simulink model "switch_inductor_system"  (R2025b)
settings: Solver=ode23t  StartTime=0.0  StopTime=10e-6  MaxStep=1e-8  RelTol=1e-4
libraries: fl_lib x93, nesl_utility x82, eeGeneralControl x28, batteryecm_lib x17, eePwmGenerator x11, slpidlib x9, simulink x2, slctrl_fre x1
(part 1 of 3)
settings Model: Creator=wjy22  LastModifiedBy=wjy22

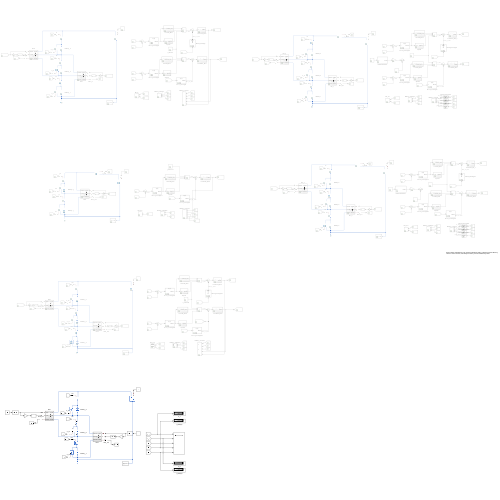
[thumbnail: Simulink's stored preview of the top-level diagram]
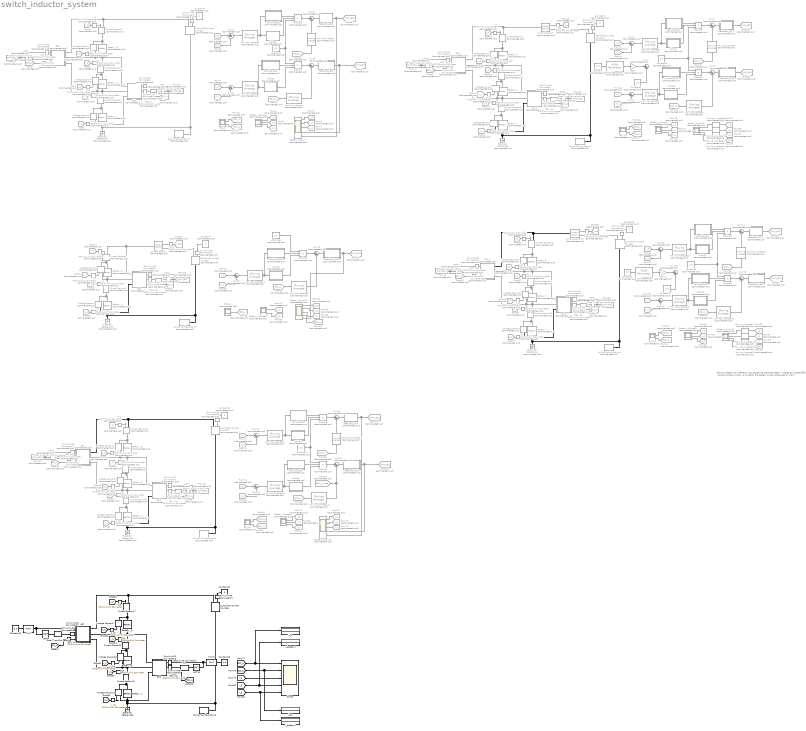
== system switch_inductor_system ==
  note: Same voltage with different inner resistance, Balance battery voltage at highest efficiency inductor current window, and satisfy the battery current scheduled by SOH.
  Alpha1 : Subsystem  Commented=on
  Alpha2 : Subsystem  Commented=on
  Alpha3 : Subsystem  Commented=on
  Alpha4 : Subsystem  Commented=on
  Alpha5 : Subsystem  Commented=on
  Alpha6 : Subsystem  Commented=on
  Alpha7 : Subsystem  Commented=on
  Alpha8 : Subsystem  Commented=on
  Alpha9 : Subsystem  Commented=on
  BC1 : Subsystem  Commented=on
  BC1_IL{,1..4} (5 alike) : nesl_utility/PS-Simulink Converter  Commented=on  PhysicalDomain=network_engine_domain  SubClassName=ps_output  LeftPortType=input  RightPortType=output  PseudoPeriodic=off  Frequencies=[]  VectorFormat=inherit  Unit=inherit  AffineConversion=off
  BC1_IL5 : nesl_utility/PS-Simulink Converter  PhysicalDomain=network_engine_domain  SubClassName=ps_output  LeftPortType=input  RightPortType=output  PseudoPeriodic=off  Frequencies=[]  VectorFormat=inherit  Unit=inherit  AffineConversion=off
  BC2 : Subsystem  Commented=on
  BC2_IL{,1..3} (4 alike) : nesl_utility/PS-Simulink Converter  Commented=on  PhysicalDomain=network_engine_domain  SubClassName=ps_output  LeftPortType=input  RightPortType=output  PseudoPeriodic=off  Frequencies=[]  VectorFormat=inherit  Unit=inherit  AffineConversion=off
  BC2_IL4 : nesl_utility/PS-Simulink Converter  PhysicalDomain=network_engine_domain  SubClassName=ps_output  LeftPortType=input  RightPortType=output  PseudoPeriodic=off  Frequencies=[]  VectorFormat=inherit  Unit=inherit  AffineConversion=off
  BC3 : Subsystem  Commented=on
  BC4 : Subsystem  Commented=on
  BC5 : Subsystem  Commented=on
  BC6 : Subsystem
  BC7 : Subsystem
  BC_1 : Subsystem  Commented=on
  BC_2 : Subsystem  Commented=on
  BC_3 : Subsystem  Commented=on
  BC_4 : Subsystem  Commented=on
  BC_IL{,1,3..4} (4 alike) : Scope  Commented=on  NumInputPorts=2
      BC_IL settings: ActiveDisplayYMinimum=0.30113223762513219  ActiveDisplayYMaximum=0.30789063396141053  DataLoggingVariableName=ScopeData4
      BC_IL1 settings: ActiveDisplayYMinimum=-0.37448035272574393  ActiveDisplayYMaximum=-0.29986535447261758
      BC_IL3 settings: ActiveDisplayYMinimum=-0.37448035272574393  ActiveDisplayYMaximum=-0.29986535447261758  DataLoggingVariableName=ScopeData14
      BC_IL4 settings: ActiveDisplayYMinimum=0.30113223762513219  ActiveDisplayYMaximum=0.30789063396141053  DataLoggingVariableName=ScopeData17
  BC_IL2 : Scope  Commented=on
      settings: ActiveDisplayYMinimum=-0.43402408027628592  ActiveDisplayYMaximum=0.45876699221950035  DataLoggingVariableName=ScopeData6
  Battery 1 : batteryecm_lib/Battery  Commented=on  Vnom=4.2 V  prm_dir=simscape.enum.battery.prm_dir.disabled  R1_dis=2 Ohm  R1_ch=2 Ohm  R1=0.0075 Ohm  prm_AH=simscape.enum.battery.prm_AH.finite  AH=0.0026 A*hr  V1=3.7 V  AH1=0.00143 A*hr  prm_R2=simscape.enum.battery.prm_R2.disabled  R2=2000 Ohm  Tmeas=298.15 K  charge_measurement_port=simscape.enum.battery.enable.no  prm_dyn=simscape.enum.battery.prm_dyn.off  Rp1=0.005 Ohm  tau1=30 s  Rp2=0.005 Ohm  tau2=30 s  Rp3=0.005 Ohm  tau3=30 s  Rp4=0.005 Ohm  tau4=30 s  Rp5=0.005 Ohm  tau5=30 s  prm_fade=simscape.enum.battery.prm_fade.disabled  N_fade=100  AH_fade=45 A*hr  R1_fade=2.02 Ohm  R1_ch_fade=2.02 Ohm  V1_fade=10.35 V  prm_age=simscape.enum.battery.prm_age.disabled  prm_age_OCV=simscape.enum.battery.prm_age_OCV.OCV  OCV_age=0.9  SOC_age=60  Tmeas_age=298.15 K  delta_time_age_vec=[0] d  temperature_age_vec=[273] K  OCV_scaling_age=2.2134e6  OCV_offset_age=1.632e6  temp_exp_age=0.515833569 V  t_exp_age=0.75  Vnom_T2=12 V  R1_T2=2.2 Ohm  R1_T2_dis=2.2 Ohm  R1_T2_ch=2.2 Ohm  V1_T2=11.4 V  R2_T2=2200 Ohm  Rp1_T2=0.005 Ohm  tau1_T2=30 s  Rp2_T2=0.005 Ohm  tau2_T2=30 s  Rp3_T2=0.005 Ohm  tau3_T2=30 s  Rp4_T2=0.005 Ohm  tau4_T2=30 s  Rp5_T2=0.005 Ohm  tau5_T2=30 s  Tmeas2=273.15 K  thermal_port=simscape.enum.thermaleffects.omit  thermal_mass=30000 J/K  i_specify=off  i_priority=None  i=0 A  i_nominal_specify=off  i_nominal_value=1  i_nominal_unit=A  v_specify=on  v_priority=High  v=3.8 V  v_nominal_specify=off  v_nominal_value=1  v_nominal_unit=V  charge_specify=on  charge_priority=None  charge=0.001072 A*hr  charge_nominal_specify=off  charge_nominal_value=1  charge_nominal_unit=A*hr  num_cycles_specify=off  num_cycles_priority=High  num_cycles=0  num_cycles_nominal_specify=off  num_cycles_nominal_value=1  num_cycles_nominal_unit=1  temperature_specify=off  temperature_priority=High  temperature=298.15 K  temperature_nominal_specify=off  temperature_nominal_value=1  temperature_nominal_unit=K
      settings: LibrarySourceBlock=batt_lib/Cells/Battery
  Battery 1_ : batteryecm_lib/Battery  Commented=on  Vnom=4.2 V  prm_dir=simscape.enum.battery.prm_dir.disabled  R1_dis=2 Ohm  R1_ch=2 Ohm  R1=0.0065 Ohm  prm_AH=simscape.enum.battery.prm_AH.finite  AH=0.0026 A*hr  V1=3.7 V  AH1=0.00143 A*hr  prm_R2=simscape.enum.battery.prm_R2.disabled  R2=2000 Ohm  Tmeas=298.15 K  charge_measurement_port=simscape.enum.battery.enable.no  prm_dyn=simscape.enum.battery.prm_dyn.off  Rp1=0.005 Ohm  tau1=30 s  Rp2=0.005 Ohm  tau2=30 s  Rp3=0.005 Ohm  tau3=30 s  Rp4=0.005 Ohm  tau4=30 s  Rp5=0.005 Ohm  tau5=30 s  prm_fade=simscape.enum.battery.prm_fade.disabled  N_fade=100  AH_fade=45 A*hr  R1_fade=2.02 Ohm  R1_ch_fade=2.02 Ohm  V1_fade=10.35 V  prm_age=simscape.enum.battery.prm_age.disabled  prm_age_OCV=simscape.enum.battery.prm_age_OCV.OCV  OCV_age=0.9  SOC_age=60  Tmeas_age=298.15 K  delta_time_age_vec=[0] d  temperature_age_vec=[273] K  OCV_scaling_age=2.2134e6  OCV_offset_age=1.632e6  temp_exp_age=0.515833569 V  t_exp_age=0.75  Vnom_T2=12 V  R1_T2=2.2 Ohm  R1_T2_dis=2.2 Ohm  R1_T2_ch=2.2 Ohm  V1_T2=11.4 V  R2_T2=2200 Ohm  Rp1_T2=0.005 Ohm  tau1_T2=30 s  Rp2_T2=0.005 Ohm  tau2_T2=30 s  Rp3_T2=0.005 Ohm  tau3_T2=30 s  Rp4_T2=0.005 Ohm  tau4_T2=30 s  Rp5_T2=0.005 Ohm  tau5_T2=30 s  Tmeas2=273.15 K  thermal_port=simscape.enum.thermaleffects.omit  thermal_mass=30000 J/K  i_specify=off  i_priority=None  i=0 A  i_nominal_specify=off  i_nominal_value=1  i_nominal_unit=A  v_specify=on  v_priority=High  v=4 V  v_nominal_specify=off  v_nominal_value=1  v_nominal_unit=V  charge_specify=on  charge_priority=None  charge=0.001072 A*hr  charge_nominal_specify=off  charge_nominal_value=1  charge_nominal_unit=A*hr  num_cycles_specify=off  num_cycles_priority=High  num_cycles=0  num_cycles_nominal_specify=off  num_cycles_nominal_value=1  num_cycles_nominal_unit=1  temperature_specify=off  temperature_priority=High  temperature=298.15 K  temperature_nominal_specify=off  temperature_nominal_value=1  temperature_nominal_unit=K
      settings: LibrarySourceBlock=batt_lib/Cells/Battery
  Battery 2 : batteryecm_lib/Battery  Commented=on  Vnom=4.2 V  prm_dir=simscape.enum.battery.prm_dir.disabled  R1_dis=2 Ohm  R1_ch=2 Ohm  R1=0.0065 Ohm  prm_AH=simscape.enum.battery.prm_AH.finite  AH=0.0026 A*hr  V1=3.7 V  AH1=0.00143 A*hr  prm_R2=simscape.enum.battery.prm_R2.disabled  R2=2000 Ohm  Tmeas=298.15 K  charge_measurement_port=simscape.enum.battery.enable.no  prm_dyn=simscape.enum.battery.prm_dyn.off  Rp1=0.005 Ohm  tau1=30 s  Rp2=0.005 Ohm  tau2=30 s  Rp3=0.005 Ohm  tau3=30 s  Rp4=0.005 Ohm  tau4=30 s  Rp5=0.005 Ohm  tau5=30 s  prm_fade=simscape.enum.battery.prm_fade.disabled  N_fade=100  AH_fade=45 A*hr  R1_fade=2.02 Ohm  R1_ch_fade=2.02 Ohm  V1_fade=10.35 V  prm_age=simscape.enum.battery.prm_age.disabled  prm_age_OCV=simscape.enum.battery.prm_age_OCV.OCV  OCV_age=0.9  SOC_age=60  Tmeas_age=298.15 K  delta_time_age_vec=[0] d  temperature_age_vec=[273] K  OCV_scaling_age=2.2134e6  OCV_offset_age=1.632e6  temp_exp_age=0.515833569 V  t_exp_age=0.75  Vnom_T2=12 V  R1_T2=2.2 Ohm  R1_T2_dis=2.2 Ohm  R1_T2_ch=2.2 Ohm  V1_T2=11.4 V  R2_T2=2200 Ohm  Rp1_T2=0.005 Ohm  tau1_T2=30 s  Rp2_T2=0.005 Ohm  tau2_T2=30 s  Rp3_T2=0.005 Ohm  tau3_T2=30 s  Rp4_T2=0.005 Ohm  tau4_T2=30 s  Rp5_T2=0.005 Ohm  tau5_T2=30 s  Tmeas2=273.15 K  thermal_port=simscape.enum.thermaleffects.omit  thermal_mass=30000 J/K  i_specify=off  i_priority=None  i=0 A  i_nominal_specify=off  i_nominal_value=1  i_nominal_unit=A  v_specify=on  v_priority=High  v=4 V  v_nominal_specify=off  v_nominal_value=1  v_nominal_unit=V  charge_specify=on  charge_priority=None  charge=0.001588 A*hr  charge_nominal_specify=off  charge_nominal_value=1  charge_nominal_unit=A*hr  num_cycles_specify=off  num_cycles_priority=High  num_cycles=0  num_cycles_nominal_specify=off  num_cycles_nominal_value=1  num_cycles_nominal_unit=1  temperature_specify=off  temperature_priority=High  temperature=298.15 K  temperature_nominal_specify=off  temperature_nominal_value=1  temperature_nominal_unit=K
      settings: LibrarySourceBlock=batt_lib/Cells/Battery
  Battery 2_ : batteryecm_lib/Battery  Commented=on  Vnom=4.2 V  prm_dir=simscape.enum.battery.prm_dir.disabled  R1_dis=2 Ohm  R1_ch=2 Ohm  R1=0.0065 Ohm  prm_AH=simscape.enum.battery.prm_AH.finite  AH=0.0026 A*hr  V1=3.7 V  AH1=0.00143 A*hr  prm_R2=simscape.enum.battery.prm_R2.disabled  R2=2000 Ohm  Tmeas=298.15 K  charge_measurement_port=simscape.enum.battery.enable.no  prm_dyn=simscape.enum.battery.prm_dyn.off  Rp1=0.005 Ohm  tau1=30 s  Rp2=0.005 Ohm  tau2=30 s  Rp3=0.005 Ohm  tau3=30 s  Rp4=0.005 Ohm  tau4=30 s  Rp5=0.005 Ohm  tau5=30 s  prm_fade=simscape.enum.battery.prm_fade.disabled  N_fade=100  AH_fade=45 A*hr  R1_fade=2.02 Ohm  R1_ch_fade=2.02 Ohm  V1_fade=10.35 V  prm_age=simscape.enum.battery.prm_age.disabled  prm_age_OCV=simscape.enum.battery.prm_age_OCV.OCV  OCV_age=0.9  SOC_age=60  Tmeas_age=298.15 K  delta_time_age_vec=[0] d  temperature_age_vec=[273] K  OCV_scaling_age=2.2134e6  OCV_offset_age=1.632e6  temp_exp_age=0.515833569 V  t_exp_age=0.75  Vnom_T2=12 V  R1_T2=2.2 Ohm  R1_T2_dis=2.2 Ohm  R1_T2_ch=2.2 Ohm  V1_T2=11.4 V  R2_T2=2200 Ohm  Rp1_T2=0.005 Ohm  tau1_T2=30 s  Rp2_T2=0.005 Ohm  tau2_T2=30 s  Rp3_T2=0.005 Ohm  tau3_T2=30 s  Rp4_T2=0.005 Ohm  tau4_T2=30 s  Rp5_T2=0.005 Ohm  tau5_T2=30 s  Tmeas2=273.15 K  thermal_port=simscape.enum.thermaleffects.omit  thermal_mass=30000 J/K  i_specify=off  i_priority=None  i=0 A  i_nominal_specify=off  i_nominal_value=1  i_nominal_unit=A  v_specify=on  v_priority=High  v=4.2 V  v_nominal_specify=off  v_nominal_value=1  v_nominal_unit=V  charge_specify=on  charge_priority=None  charge=0.001588 A*hr  charge_nominal_specify=off  charge_nominal_value=1  charge_nominal_unit=A*hr  num_cycles_specify=off  num_cycles_priority=High  num_cycles=0  num_cycles_nominal_specify=off  num_cycles_nominal_value=1  num_cycles_nominal_unit=1  temperature_specify=off  temperature_priority=High  temperature=298.15 K  temperature_nominal_specify=off  temperature_nominal_value=1  temperature_nominal_unit=K
      settings: LibrarySourceBlock=batt_lib/Cells/Battery
  Battery 3 : batteryecm_lib/Battery  Commented=on  Vnom=4.2 V  prm_dir=simscape.enum.battery.prm_dir.disabled  R1_dis=2 Ohm  R1_ch=2 Ohm  R1=0.005 Ohm  prm_AH=simscape.enum.battery.prm_AH.finite  AH=0.0026 A*hr  V1=3.7 V  AH1=0.00143 A*hr  prm_R2=simscape.enum.battery.prm_R2.disabled  R2=2000 Ohm  Tmeas=298.15 K  charge_measurement_port=simscape.enum.battery.enable.no  prm_dyn=simscape.enum.battery.prm_dyn.off  Rp1=0.005 Ohm  tau1=30 s  Rp2=0.005 Ohm  tau2=30 s  Rp3=0.005 Ohm  tau3=30 s  Rp4=0.005 Ohm  tau4=30 s  Rp5=0.005 Ohm  tau5=30 s  prm_fade=simscape.enum.battery.prm_fade.disabled  N_fade=100  AH_fade=45 A*hr  R1_fade=2.02 Ohm  R1_ch_fade=2.02 Ohm  V1_fade=10.35 V  prm_age=simscape.enum.battery.prm_age.disabled  prm_age_OCV=simscape.enum.battery.prm_age_OCV.OCV  OCV_age=0.9  SOC_age=60  Tmeas_age=298.15 K  delta_time_age_vec=[0] d  temperature_age_vec=[273] K  OCV_scaling_age=2.2134e6  OCV_offset_age=1.632e6  temp_exp_age=0.515833569 V  t_exp_age=0.75  Vnom_T2=12 V  R1_T2=2.2 Ohm  R1_T2_dis=2.2 Ohm  R1_T2_ch=2.2 Ohm  V1_T2=11.4 V  R2_T2=2200 Ohm  Rp1_T2=0.005 Ohm  tau1_T2=30 s  Rp2_T2=0.005 Ohm  tau2_T2=30 s  Rp3_T2=0.005 Ohm  tau3_T2=30 s  Rp4_T2=0.005 Ohm  tau4_T2=30 s  Rp5_T2=0.005 Ohm  tau5_T2=30 s  Tmeas2=273.15 K  thermal_port=simscape.enum.thermaleffects.omit  thermal_mass=30000 J/K  i_specify=off  i_priority=None  i=0 A  i_nominal_specify=off  i_nominal_value=1  i_nominal_unit=A  v_specify=on  v_priority=High  v=4.2 V  v_nominal_specify=off  v_nominal_value=1  v_nominal_unit=V  charge_specify=on  charge_priority=None  charge=0.0026 A*hr  charge_nominal_specify=off  charge_nominal_value=1  charge_nominal_unit=A*hr  num_cycles_specify=off  num_cycles_priority=High  num_cycles=0  num_cycles_nominal_specify=off  num_cycles_nominal_value=1  num_cycles_nominal_unit=1  temperature_specify=off  temperature_priority=High  temperature=298.15 K  temperature_nominal_specify=off  temperature_nominal_value=1  temperature_nominal_unit=K
      settings: LibrarySourceBlock=batt_lib/Cells/Battery
  Battery 4 : batteryecm_lib/Battery  Commented=on  Vnom=4.2 V  prm_dir=simscape.enum.battery.prm_dir.disabled  R1_dis=2 Ohm  R1_ch=2 Ohm  R1=0.0075 Ohm  prm_AH=simscape.enum.battery.prm_AH.finite  AH=0.0026 A*hr  V1=3.7 V  AH1=0.00143 A*hr  prm_R2=simscape.enum.battery.prm_R2.disabled  R2=2000 Ohm  Tmeas=298.15 K  charge_measurement_port=simscape.enum.battery.enable.no  prm_dyn=simscape.enum.battery.prm_dyn.off  Rp1=0.005 Ohm  tau1=30 s  Rp2=0.005 Ohm  tau2=30 s  Rp3=0.005 Ohm  tau3=30 s  Rp4=0.005 Ohm  tau4=30 s  Rp5=0.005 Ohm  tau5=30 s  prm_fade=simscape.enum.battery.prm_fade.disabled  N_fade=100  AH_fade=45 A*hr  R1_fade=2.02 Ohm  R1_ch_fade=2.02 Ohm  V1_fade=10.35 V  prm_age=simscape.enum.battery.prm_age.disabled  prm_age_OCV=simscape.enum.battery.prm_age_OCV.OCV  OCV_age=0.9  SOC_age=60  Tmeas_age=298.15 K  delta_time_age_vec=[0] d  temperature_age_vec=[273] K  OCV_scaling_age=2.2134e6  OCV_offset_age=1.632e6  temp_exp_age=0.515833569 V  t_exp_age=0.75  Vnom_T2=12 V  R1_T2=2.2 Ohm  R1_T2_dis=2.2 Ohm  R1_T2_ch=2.2 Ohm  V1_T2=11.4 V  R2_T2=2200 Ohm  Rp1_T2=0.005 Ohm  tau1_T2=30 s  Rp2_T2=0.005 Ohm  tau2_T2=30 s  Rp3_T2=0.005 Ohm  tau3_T2=30 s  Rp4_T2=0.005 Ohm  tau4_T2=30 s  Rp5_T2=0.005 Ohm  tau5_T2=30 s  Tmeas2=273.15 K  thermal_port=simscape.enum.thermaleffects.omit  thermal_mass=30000 J/K  i_specify=off  i_priority=None  i=0 A  i_nominal_specify=off  i_nominal_value=1  i_nominal_unit=A  v_specify=on  v_priority=High  v=3.8 V  v_nominal_specify=off  v_nominal_value=1  v_nominal_unit=V  charge_specify=on  charge_priority=None  charge=0.001072 A*hr  charge_nominal_specify=off  charge_nominal_value=1  charge_nominal_unit=A*hr  num_cycles_specify=off  num_cycles_priority=High  num_cycles=0  num_cycles_nominal_specify=off  num_cycles_nominal_value=1  num_cycles_nominal_unit=1  temperature_specify=off  temperature_priority=High  temperature=298.15 K  temperature_nominal_specify=off  temperature_nominal_value=1  temperature_nominal_unit=K
      settings: LibrarySourceBlock=batt_lib/Cells/Battery
  Battery 5 : batteryecm_lib/Battery  Commented=on  Vnom=4.2 V  prm_dir=simscape.enum.battery.prm_dir.disabled  R1_dis=2 Ohm  R1_ch=2 Ohm  R1=0.0065 Ohm  prm_AH=simscape.enum.battery.prm_AH.finite  AH=0.0026 A*hr  V1=3.7 V  AH1=0.00143 A*hr  prm_R2=simscape.enum.battery.prm_R2.disabled  R2=2000 Ohm  Tmeas=298.15 K  charge_measurement_port=simscape.enum.battery.enable.no  prm_dyn=simscape.enum.battery.prm_dyn.off  Rp1=0.005 Ohm  tau1=30 s  Rp2=0.005 Ohm  tau2=30 s  Rp3=0.005 Ohm  tau3=30 s  Rp4=0.005 Ohm  tau4=30 s  Rp5=0.005 Ohm  tau5=30 s  prm_fade=simscape.enum.battery.prm_fade.disabled  N_fade=100  AH_fade=45 A*hr  R1_fade=2.02 Ohm  R1_ch_fade=2.02 Ohm  V1_fade=10.35 V  prm_age=simscape.enum.battery.prm_age.disabled  prm_age_OCV=simscape.enum.battery.prm_age_OCV.OCV  OCV_age=0.9  SOC_age=60  Tmeas_age=298.15 K  delta_time_age_vec=[0] d  temperature_age_vec=[273] K  OCV_scaling_age=2.2134e6  OCV_offset_age=1.632e6  temp_exp_age=0.515833569 V  t_exp_age=0.75  Vnom_T2=12 V  R1_T2=2.2 Ohm  R1_T2_dis=2.2 Ohm  R1_T2_ch=2.2 Ohm  V1_T2=11.4 V  R2_T2=2200 Ohm  Rp1_T2=0.005 Ohm  tau1_T2=30 s  Rp2_T2=0.005 Ohm  tau2_T2=30 s  Rp3_T2=0.005 Ohm  tau3_T2=30 s  Rp4_T2=0.005 Ohm  tau4_T2=30 s  Rp5_T2=0.005 Ohm  tau5_T2=30 s  Tmeas2=273.15 K  thermal_port=simscape.enum.thermaleffects.omit  thermal_mass=30000 J/K  i_specify=off  i_priority=None  i=0 A  i_nominal_specify=off  i_nominal_value=1  i_nominal_unit=A  v_specify=on  v_priority=High  v=4 V  v_nominal_specify=off  v_nominal_value=1  v_nominal_unit=V  charge_specify=on  charge_priority=None  charge=0.001588 A*hr  charge_nominal_specify=off  charge_nominal_value=1  charge_nominal_unit=A*hr  num_cycles_specify=off  num_cycles_priority=High  num_cycles=0  num_cycles_nominal_specify=off  num_cycles_nominal_value=1  num_cycles_nominal_unit=1  temperature_specify=off  temperature_priority=High  temperature=298.15 K  temperature_nominal_specify=off  temperature_nominal_value=1  temperature_nominal_unit=K
      settings: LibrarySourceBlock=batt_lib/Cells/Battery
  Battery 6 : batteryecm_lib/Battery  Commented=on  Vnom=4.2 V  prm_dir=simscape.enum.battery.prm_dir.disabled  R1_dis=2 Ohm  R1_ch=2 Ohm  R1=0.005 Ohm  prm_AH=simscape.enum.battery.prm_AH.finite  AH=0.0026 A*hr  V1=3.7 V  AH1=0.00143 A*hr  prm_R2=simscape.enum.battery.prm_R2.disabled  R2=2000 Ohm  Tmeas=298.15 K  charge_measurement_port=simscape.enum.battery.enable.no  prm_dyn=simscape.enum.battery.prm_dyn.off  Rp1=0.005 Ohm  tau1=30 s  Rp2=0.005 Ohm  tau2=30 s  Rp3=0.005 Ohm  tau3=30 s  Rp4=0.005 Ohm  tau4=30 s  Rp5=0.005 Ohm  tau5=30 s  prm_fade=simscape.enum.battery.prm_fade.disabled  N_fade=100  AH_fade=45 A*hr  R1_fade=2.02 Ohm  R1_ch_fade=2.02 Ohm  V1_fade=10.35 V  prm_age=simscape.enum.battery.prm_age.disabled  prm_age_OCV=simscape.enum.battery.prm_age_OCV.OCV  OCV_age=0.9  SOC_age=60  Tmeas_age=298.15 K  delta_time_age_vec=[0] d  temperature_age_vec=[273] K  OCV_scaling_age=2.2134e6  OCV_offset_age=1.632e6  temp_exp_age=0.515833569 V  t_exp_age=0.75  Vnom_T2=12 V  R1_T2=2.2 Ohm  R1_T2_dis=2.2 Ohm  R1_T2_ch=2.2 Ohm  V1_T2=11.4 V  R2_T2=2200 Ohm  Rp1_T2=0.005 Ohm  tau1_T2=30 s  Rp2_T2=0.005 Ohm  tau2_T2=30 s  Rp3_T2=0.005 Ohm  tau3_T2=30 s  Rp4_T2=0.005 Ohm  tau4_T2=30 s  Rp5_T2=0.005 Ohm  tau5_T2=30 s  Tmeas2=273.15 K  thermal_port=simscape.enum.thermaleffects.omit  thermal_mass=30000 J/K  i_specify=off  i_priority=None  i=0 A  i_nominal_specify=off  i_nominal_value=1  i_nominal_unit=A  v_specify=on  v_priority=High  v=4.2 V  v_nominal_specify=off  v_nominal_value=1  v_nominal_unit=V  charge_specify=on  charge_priority=None  charge=0.0026 A*hr  charge_nominal_specify=off  charge_nominal_value=1  charge_nominal_unit=A*hr  num_cycles_specify=off  num_cycles_priority=High  num_cycles=0  num_cycles_nominal_specify=off  num_cycles_nominal_value=1  num_cycles_nominal_unit=1  temperature_specify=off  temperature_priority=High  temperature=298.15 K  temperature_nominal_specify=off  temperature_nominal_value=1  temperature_nominal_unit=K
      settings: LibrarySourceBlock=batt_lib/Cells/Battery
  Battery _1 : batteryecm_lib/Battery  Commented=on  Vnom=4.2 V  prm_dir=simscape.enum.battery.prm_dir.disabled  R1_dis=2 Ohm  R1_ch=2 Ohm  R1=0.0065 Ohm  prm_AH=simscape.enum.battery.prm_AH.finite  AH=0.0026 A*hr  V1=3.7 V  AH1=0.00143 A*hr  prm_R2=simscape.enum.battery.prm_R2.disabled  R2=2000 Ohm  Tmeas=298.15 K  charge_measurement_port=simscape.enum.battery.enable.no  prm_dyn=simscape.enum.battery.prm_dyn.off  Rp1=0.005 Ohm  tau1=30 s  Rp2=0.005 Ohm  tau2=30 s  Rp3=0.005 Ohm  tau3=30 s  Rp4=0.005 Ohm  tau4=30 s  Rp5=0.005 Ohm  tau5=30 s  prm_fade=simscape.enum.battery.prm_fade.disabled  N_fade=100  AH_fade=45 A*hr  R1_fade=2.02 Ohm  R1_ch_fade=2.02 Ohm  V1_fade=10.35 V  prm_age=simscape.enum.battery.prm_age.disabled  prm_age_OCV=simscape.enum.battery.prm_age_OCV.OCV  OCV_age=0.9  SOC_age=60  Tmeas_age=298.15 K  delta_time_age_vec=[0] d  temperature_age_vec=[273] K  OCV_scaling_age=2.2134e6  OCV_offset_age=1.632e6  temp_exp_age=0.515833569 V  t_exp_age=0.75  Vnom_T2=12 V  R1_T2=2.2 Ohm  R1_T2_dis=2.2 Ohm  R1_T2_ch=2.2 Ohm  V1_T2=11.4 V  R2_T2=2200 Ohm  Rp1_T2=0.005 Ohm  tau1_T2=30 s  Rp2_T2=0.005 Ohm  tau2_T2=30 s  Rp3_T2=0.005 Ohm  tau3_T2=30 s  Rp4_T2=0.005 Ohm  tau4_T2=30 s  Rp5_T2=0.005 Ohm  tau5_T2=30 s  Tmeas2=273.15 K  thermal_port=simscape.enum.thermaleffects.omit  thermal_mass=30000 J/K  i_specify=off  i_priority=None  i=0 A  i_nominal_specify=off  i_nominal_value=1  i_nominal_unit=A  v_specify=on  v_priority=High  v=4 V  v_nominal_specify=off  v_nominal_value=1  v_nominal_unit=V  charge_specify=on  charge_priority=None  charge=0.001072 A*hr  charge_nominal_specify=off  charge_nominal_value=1  charge_nominal_unit=A*hr  num_cycles_specify=off  num_cycles_priority=High  num_cycles=0  num_cycles_nominal_specify=off  num_cycles_nominal_value=1  num_cycles_nominal_unit=1  temperature_specify=off  temperature_priority=High  temperature=298.15 K  temperature_nominal_specify=off  temperature_nominal_value=1  temperature_nominal_unit=K
      settings: LibrarySourceBlock=batt_lib/Cells/Battery
  Battery _2 : batteryecm_lib/Battery  Commented=on  Vnom=4.2 V  prm_dir=simscape.enum.battery.prm_dir.disabled  R1_dis=2 Ohm  R1_ch=2 Ohm  R1=0.0065 Ohm  prm_AH=simscape.enum.battery.prm_AH.finite  AH=0.0026 A*hr  V1=3.7 V  AH1=0.00143 A*hr  prm_R2=simscape.enum.battery.prm_R2.disabled  R2=2000 Ohm  Tmeas=298.15 K  charge_measurement_port=simscape.enum.battery.enable.no  prm_dyn=simscape.enum.battery.prm_dyn.off  Rp1=0.005 Ohm  tau1=30 s  Rp2=0.005 Ohm  tau2=30 s  Rp3=0.005 Ohm  tau3=30 s  Rp4=0.005 Ohm  tau4=30 s  Rp5=0.005 Ohm  tau5=30 s  prm_fade=simscape.enum.battery.prm_fade.disabled  N_fade=100  AH_fade=45 A*hr  R1_fade=2.02 Ohm  R1_ch_fade=2.02 Ohm  V1_fade=10.35 V  prm_age=simscape.enum.battery.prm_age.disabled  prm_age_OCV=simscape.enum.battery.prm_age_OCV.OCV  OCV_age=0.9  SOC_age=60  Tmeas_age=298.15 K  delta_time_age_vec=[0] d  temperature_age_vec=[273] K  OCV_scaling_age=2.2134e6  OCV_offset_age=1.632e6  temp_exp_age=0.515833569 V  t_exp_age=0.75  Vnom_T2=12 V  R1_T2=2.2 Ohm  R1_T2_dis=2.2 Ohm  R1_T2_ch=2.2 Ohm  V1_T2=11.4 V  R2_T2=2200 Ohm  Rp1_T2=0.005 Ohm  tau1_T2=30 s  Rp2_T2=0.005 Ohm  tau2_T2=30 s  Rp3_T2=0.005 Ohm  tau3_T2=30 s  Rp4_T2=0.005 Ohm  tau4_T2=30 s  Rp5_T2=0.005 Ohm  tau5_T2=30 s  Tmeas2=273.15 K  thermal_port=simscape.enum.thermaleffects.omit  thermal_mass=30000 J/K  i_specify=off  i_priority=None  i=0 A  i_nominal_specify=off  i_nominal_value=1  i_nominal_unit=A  v_specify=on  v_priority=High  v=4.2 V  v_nominal_specify=off  v_nominal_value=1  v_nominal_unit=V  charge_specify=on  charge_priority=None  charge=0.001588 A*hr  charge_nominal_specify=off  charge_nominal_value=1  charge_nominal_unit=A*hr  num_cycles_specify=off  num_cycles_priority=High  num_cycles=0  num_cycles_nominal_specify=off  num_cycles_nominal_value=1  num_cycles_nominal_unit=1  temperature_specify=off  temperature_priority=High  temperature=298.15 K  temperature_nominal_specify=off  temperature_nominal_value=1  temperature_nominal_unit=K
      settings: LibrarySourceBlock=batt_lib/Cells/Battery
  Battery _3 : batteryecm_lib/Battery  Commented=on  Vnom=4.2 V  prm_dir=simscape.enum.battery.prm_dir.disabled  R1_dis=2 Ohm  R1_ch=2 Ohm  R1=0.0065 Ohm  prm_AH=simscape.enum.battery.prm_AH.finite  AH=0.0026 A*hr  V1=3.7 V  AH1=0.00143 A*hr  prm_R2=simscape.enum.battery.prm_R2.disabled  R2=2000 Ohm  Tmeas=298.15 K  charge_measurement_port=simscape.enum.battery.enable.no  prm_dyn=simscape.enum.battery.prm_dyn.off  Rp1=0.005 Ohm  tau1=30 s  Rp2=0.005 Ohm  tau2=30 s  Rp3=0.005 Ohm  tau3=30 s  Rp4=0.005 Ohm  tau4=30 s  Rp5=0.005 Ohm  tau5=30 s  prm_fade=simscape.enum.battery.prm_fade.disabled  N_fade=100  AH_fade=45 A*hr  R1_fade=2.02 Ohm  R1_ch_fade=2.02 Ohm  V1_fade=10.35 V  prm_age=simscape.enum.battery.prm_age.disabled  prm_age_OCV=simscape.enum.battery.prm_age_OCV.OCV  OCV_age=0.9  SOC_age=60  Tmeas_age=298.15 K  delta_time_age_vec=[0] d  temperature_age_vec=[273] K  OCV_scaling_age=2.2134e6  OCV_offset_age=1.632e6  temp_exp_age=0.515833569 V  t_exp_age=0.75  Vnom_T2=12 V  R1_T2=2.2 Ohm  R1_T2_dis=2.2 Ohm  R1_T2_ch=2.2 Ohm  V1_T2=11.4 V  R2_T2=2200 Ohm  Rp1_T2=0.005 Ohm  tau1_T2=30 s  Rp2_T2=0.005 Ohm  tau2_T2=30 s  Rp3_T2=0.005 Ohm  tau3_T2=30 s  Rp4_T2=0.005 Ohm  tau4_T2=30 s  Rp5_T2=0.005 Ohm  tau5_T2=30 s  Tmeas2=273.15 K  thermal_port=simscape.enum.thermaleffects.omit  thermal_mass=30000 J/K  i_specify=off  i_priority=None  i=0 A  i_nominal_specify=off  i_nominal_value=1  i_nominal_unit=A  v_specify=on  v_priority=High  v=3.8 V  v_nominal_specify=off  v_nominal_value=1  v_nominal_unit=V  charge_specify=on  charge_priority=None  charge=0.0026 A*hr  charge_nominal_specify=off  charge_nominal_value=1  charge_nominal_unit=A*hr  num_cycles_specify=off  num_cycles_priority=High  num_cycles=0  num_cycles_nominal_specify=off  num_cycles_nominal_value=1  num_cycles_nominal_unit=1  temperature_specify=off  temperature_priority=High  temperature=298.15 K  temperature_nominal_specify=off  temperature_nominal_value=1  temperature_nominal_unit=K
      settings: LibrarySourceBlock=batt_lib/Cells/Battery
  Battery _4 : batteryecm_lib/Battery  Commented=on  Vnom=4.2 V  prm_dir=simscape.enum.battery.prm_dir.disabled  R1_dis=2 Ohm  R1_ch=2 Ohm  R1=0.0065 Ohm  prm_AH=simscape.enum.battery.prm_AH.finite  AH=0.0026 A*hr  V1=3.7 V  AH1=0.00143 A*hr  prm_R2=simscape.enum.battery.prm_R2.disabled  R2=2000 Ohm  Tmeas=298.15 K  charge_measurement_port=simscape.enum.battery.enable.no  prm_dyn=simscape.enum.battery.prm_dyn.off  Rp1=0.005 Ohm  tau1=30 s  Rp2=0.005 Ohm  tau2=30 s  Rp3=0.005 Ohm  tau3=30 s  Rp4=0.005 Ohm  tau4=30 s  Rp5=0.005 Ohm  tau5=30 s  prm_fade=simscape.enum.battery.prm_fade.disabled  N_fade=100  AH_fade=45 A*hr  R1_fade=2.02 Ohm  R1_ch_fade=2.02 Ohm  V1_fade=10.35 V  prm_age=simscape.enum.battery.prm_age.disabled  prm_age_OCV=simscape.enum.battery.prm_age_OCV.OCV  OCV_age=0.9  SOC_age=60  Tmeas_age=298.15 K  delta_time_age_vec=[0] d  temperature_age_vec=[273] K  OCV_scaling_age=2.2134e6  OCV_offset_age=1.632e6  temp_exp_age=0.515833569 V  t_exp_age=0.75  Vnom_T2=12 V  R1_T2=2.2 Ohm  R1_T2_dis=2.2 Ohm  R1_T2_ch=2.2 Ohm  V1_T2=11.4 V  R2_T2=2200 Ohm  Rp1_T2=0.005 Ohm  tau1_T2=30 s  Rp2_T2=0.005 Ohm  tau2_T2=30 s  Rp3_T2=0.005 Ohm  tau3_T2=30 s  Rp4_T2=0.005 Ohm  tau4_T2=30 s  Rp5_T2=0.005 Ohm  tau5_T2=30 s  Tmeas2=273.15 K  thermal_port=simscape.enum.thermaleffects.omit  thermal_mass=30000 J/K  i_specify=off  i_priority=None  i=0 A  i_nominal_specify=off  i_nominal_value=1  i_nominal_unit=A  v_specify=on  v_priority=High  v=4 V  v_nominal_specify=off  v_nominal_value=1  v_nominal_unit=V  charge_specify=on  charge_priority=None  charge=0.001072 A*hr  charge_nominal_specify=off  charge_nominal_value=1  charge_nominal_unit=A*hr  num_cycles_specify=off  num_cycles_priority=High  num_cycles=0  num_cycles_nominal_specify=off  num_cycles_nominal_value=1  num_cycles_nominal_unit=1  temperature_specify=off  temperature_priority=High  temperature=298.15 K  temperature_nominal_specify=off  temperature_nominal_value=1  temperature_nominal_unit=K
      settings: LibrarySourceBlock=batt_lib/Cells/Battery
  Battery _5 : batteryecm_lib/Battery  Commented=on  Vnom=4.2 V  prm_dir=simscape.enum.battery.prm_dir.disabled  R1_dis=2 Ohm  R1_ch=2 Ohm  R1=0.0065 Ohm  prm_AH=simscape.enum.battery.prm_AH.finite  AH=0.0026 A*hr  V1=3.7 V  AH1=0.00143 A*hr  prm_R2=simscape.enum.battery.prm_R2.disabled  R2=2000 Ohm  Tmeas=298.15 K  charge_measurement_port=simscape.enum.battery.enable.no  prm_dyn=simscape.enum.battery.prm_dyn.off  Rp1=0.005 Ohm  tau1=30 s  Rp2=0.005 Ohm  tau2=30 s  Rp3=0.005 Ohm  tau3=30 s  Rp4=0.005 Ohm  tau4=30 s  Rp5=0.005 Ohm  tau5=30 s  prm_fade=simscape.enum.battery.prm_fade.disabled  N_fade=100  AH_fade=45 A*hr  R1_fade=2.02 Ohm  R1_ch_fade=2.02 Ohm  V1_fade=10.35 V  prm_age=simscape.enum.battery.prm_age.disabled  prm_age_OCV=simscape.enum.battery.prm_age_OCV.OCV  OCV_age=0.9  SOC_age=60  Tmeas_age=298.15 K  delta_time_age_vec=[0] d  temperature_age_vec=[273] K  OCV_scaling_age=2.2134e6  OCV_offset_age=1.632e6  temp_exp_age=0.515833569 V  t_exp_age=0.75  Vnom_T2=12 V  R1_T2=2.2 Ohm  R1_T2_dis=2.2 Ohm  R1_T2_ch=2.2 Ohm  V1_T2=11.4 V  R2_T2=2200 Ohm  Rp1_T2=0.005 Ohm  tau1_T2=30 s  Rp2_T2=0.005 Ohm  tau2_T2=30 s  Rp3_T2=0.005 Ohm  tau3_T2=30 s  Rp4_T2=0.005 Ohm  tau4_T2=30 s  Rp5_T2=0.005 Ohm  tau5_T2=30 s  Tmeas2=273.15 K  thermal_port=simscape.enum.thermaleffects.omit  thermal_mass=30000 J/K  i_specify=off  i_priority=None  i=0 A  i_nominal_specify=off  i_nominal_value=1  i_nominal_unit=A  v_specify=on  v_priority=High  v=4.2 V  v_nominal_specify=off  v_nominal_value=1  v_nominal_unit=V  charge_specify=on  charge_priority=None  charge=0.001588 A*hr  charge_nominal_specify=off  charge_nominal_value=1  charge_nominal_unit=A*hr  num_cycles_specify=off  num_cycles_priority=High  num_cycles=0  num_cycles_nominal_specify=off  num_cycles_nominal_value=1  num_cycles_nominal_unit=1  temperature_specify=off  temperature_priority=High  temperature=298.15 K  temperature_nominal_specify=off  temperature_nominal_value=1  temperature_nominal_unit=K
      settings: LibrarySourceBlock=batt_lib/Cells/Battery
  Battery _6 : batteryecm_lib/Battery  Commented=on  Vnom=4.2 V  prm_dir=simscape.enum.battery.prm_dir.disabled  R1_dis=2 Ohm  R1_ch=2 Ohm  R1=0.0065 Ohm  prm_AH=simscape.enum.battery.prm_AH.finite  AH=0.0026 A*hr  V1=3.7 V  AH1=0.00143 A*hr  prm_R2=simscape.enum.battery.prm_R2.disabled  R2=2000 Ohm  Tmeas=298.15 K  charge_measurement_port=simscape.enum.battery.enable.no  prm_dyn=simscape.enum.battery.prm_dyn.off  Rp1=0.005 Ohm  tau1=30 s  Rp2=0.005 Ohm  tau2=30 s  Rp3=0.005 Ohm  tau3=30 s  Rp4=0.005 Ohm  tau4=30 s  Rp5=0.005 Ohm  tau5=30 s  prm_fade=simscape.enum.battery.prm_fade.disabled  N_fade=100  AH_fade=45 A*hr  R1_fade=2.02 Ohm  R1_ch_fade=2.02 Ohm  V1_fade=10.35 V  prm_age=simscape.enum.battery.prm_age.disabled  prm_age_OCV=simscape.enum.battery.prm_age_OCV.OCV  OCV_age=0.9  SOC_age=60  Tmeas_age=298.15 K  delta_time_age_vec=[0] d  temperature_age_vec=[273] K  OCV_scaling_age=2.2134e6  OCV_offset_age=1.632e6  temp_exp_age=0.515833569 V  t_exp_age=0.75  Vnom_T2=12 V  R1_T2=2.2 Ohm  R1_T2_dis=2.2 Ohm  R1_T2_ch=2.2 Ohm  V1_T2=11.4 V  R2_T2=2200 Ohm  Rp1_T2=0.005 Ohm  tau1_T2=30 s  Rp2_T2=0.005 Ohm  tau2_T2=30 s  Rp3_T2=0.005 Ohm  tau3_T2=30 s  Rp4_T2=0.005 Ohm  tau4_T2=30 s  Rp5_T2=0.005 Ohm  tau5_T2=30 s  Tmeas2=273.15 K  thermal_port=simscape.enum.thermaleffects.omit  thermal_mass=30000 J/K  i_specify=off  i_priority=None  i=0 A  i_nominal_specify=off  i_nominal_value=1  i_nominal_unit=A  v_specify=on  v_priority=High  v=3.8 V  v_nominal_specify=off  v_nominal_value=1  v_nominal_unit=V  charge_specify=on  charge_priority=None  charge=0.0026 A*hr  charge_nominal_specify=off  charge_nominal_value=1  charge_nominal_unit=A*hr  num_cycles_specify=off  num_cycles_priority=High  num_cycles=0  num_cycles_nominal_specify=off  num_cycles_nominal_value=1  num_cycles_nominal_unit=1  temperature_specify=off  temperature_priority=High  temperature=298.15 K  temperature_nominal_specify=off  temperature_nominal_value=1  temperature_nominal_unit=K
      settings: LibrarySourceBlock=batt_lib/Cells/Battery
  Battery _7 : batteryecm_lib/Battery  Vnom=4.2 V  prm_dir=simscape.enum.battery.prm_dir.disabled  R1_dis=2 Ohm  R1_ch=2 Ohm  R1=0.0065 Ohm  prm_AH=simscape.enum.battery.prm_AH.finite  AH=0.0026 A*hr  V1=3.7 V  AH1=0.00143 A*hr  prm_R2=simscape.enum.battery.prm_R2.disabled  R2=2000 Ohm  Tmeas=298.15 K  charge_measurement_port=simscape.enum.battery.enable.no  prm_dyn=simscape.enum.battery.prm_dyn.off  Rp1=0.005 Ohm  tau1=30 s  Rp2=0.005 Ohm  tau2=30 s  Rp3=0.005 Ohm  tau3=30 s  Rp4=0.005 Ohm  tau4=30 s  Rp5=0.005 Ohm  tau5=30 s  prm_fade=simscape.enum.battery.prm_fade.disabled  N_fade=100  AH_fade=45 A*hr  R1_fade=2.02 Ohm  R1_ch_fade=2.02 Ohm  V1_fade=10.35 V  prm_age=simscape.enum.battery.prm_age.disabled  prm_age_OCV=simscape.enum.battery.prm_age_OCV.OCV  OCV_age=0.9  SOC_age=60  Tmeas_age=298.15 K  delta_time_age_vec=[0] d  temperature_age_vec=[273] K  OCV_scaling_age=2.2134e6  OCV_offset_age=1.632e6  temp_exp_age=0.515833569 V  t_exp_age=0.75  Vnom_T2=12 V  R1_T2=2.2 Ohm  R1_T2_dis=2.2 Ohm  R1_T2_ch=2.2 Ohm  V1_T2=11.4 V  R2_T2=2200 Ohm  Rp1_T2=0.005 Ohm  tau1_T2=30 s  Rp2_T2=0.005 Ohm  tau2_T2=30 s  Rp3_T2=0.005 Ohm  tau3_T2=30 s  Rp4_T2=0.005 Ohm  tau4_T2=30 s  Rp5_T2=0.005 Ohm  tau5_T2=30 s  Tmeas2=273.15 K  thermal_port=simscape.enum.thermaleffects.omit  thermal_mass=30000 J/K  i_specify=off  i_priority=None  i=0 A  i_nominal_specify=off  i_nominal_value=1  i_nominal_unit=A  v_specify=on  v_priority=High  v=4 V  v_nominal_specify=off  v_nominal_value=1  v_nominal_unit=V  charge_specify=on  charge_priority=None  charge=0.001072 A*hr  charge_nominal_specify=off  charge_nominal_value=1  charge_nominal_unit=A*hr  num_cycles_specify=off  num_cycles_priority=High  num_cycles=0  num_cycles_nominal_specify=off  num_cycles_nominal_value=1  num_cycles_nominal_unit=1  temperature_specify=off  temperature_priority=High  temperature=298.15 K  temperature_nominal_specify=off  temperature_nominal_value=1  temperature_nominal_unit=K
      settings: LibrarySourceBlock=batt_lib/Cells/Battery
  Battery _8 : batteryecm_lib/Battery  Vnom=4.2 V  prm_dir=simscape.enum.battery.prm_dir.disabled  R1_dis=2 Ohm  R1_ch=2 Ohm  R1=0.0065 Ohm  prm_AH=simscape.enum.battery.prm_AH.finite  AH=0.0026 A*hr  V1=3.7 V  AH1=0.00143 A*hr  prm_R2=simscape.enum.battery.prm_R2.disabled  R2=2000 Ohm  Tmeas=298.15 K  charge_measurement_port=simscape.enum.battery.enable.no  prm_dyn=simscape.enum.battery.prm_dyn.off  Rp1=0.005 Ohm  tau1=30 s  Rp2=0.005 Ohm  tau2=30 s  Rp3=0.005 Ohm  tau3=30 s  Rp4=0.005 Ohm  tau4=30 s  Rp5=0.005 Ohm  tau5=30 s  prm_fade=simscape.enum.battery.prm_fade.disabled  N_fade=100  AH_fade=45 A*hr  R1_fade=2.02 Ohm  R1_ch_fade=2.02 Ohm  V1_fade=10.35 V  prm_age=simscape.enum.battery.prm_age.disabled  prm_age_OCV=simscape.enum.battery.prm_age_OCV.OCV  OCV_age=0.9  SOC_age=60  Tmeas_age=298.15 K  delta_time_age_vec=[0] d  temperature_age_vec=[273] K  OCV_scaling_age=2.2134e6  OCV_offset_age=1.632e6  temp_exp_age=0.515833569 V  t_exp_age=0.75  Vnom_T2=12 V  R1_T2=2.2 Ohm  R1_T2_dis=2.2 Ohm  R1_T2_ch=2.2 Ohm  V1_T2=11.4 V  R2_T2=2200 Ohm  Rp1_T2=0.005 Ohm  tau1_T2=30 s  Rp2_T2=0.005 Ohm  tau2_T2=30 s  Rp3_T2=0.005 Ohm  tau3_T2=30 s  Rp4_T2=0.005 Ohm  tau4_T2=30 s  Rp5_T2=0.005 Ohm  tau5_T2=30 s  Tmeas2=273.15 K  thermal_port=simscape.enum.thermaleffects.omit  thermal_mass=30000 J/K  i_specify=off  i_priority=None  i=0 A  i_nominal_specify=off  i_nominal_value=1  i_nominal_unit=A  v_specify=on  v_priority=High  v=4.2 V  v_nominal_specify=off  v_nominal_value=1  v_nominal_unit=V  charge_specify=on  charge_priority=None  charge=0.001588 A*hr  charge_nominal_specify=off  charge_nominal_value=1  charge_nominal_unit=A*hr  num_cycles_specify=off  num_cycles_priority=High  num_cycles=0  num_cycles_nominal_specify=off  num_cycles_nominal_value=1  num_cycles_nominal_unit=1  temperature_specify=off  temperature_priority=High  temperature=298.15 K  temperature_nominal_specify=off  temperature_nominal_value=1  temperature_nominal_unit=K
      settings: LibrarySourceBlock=batt_lib/Cells/Battery
  Battery _9 : batteryecm_lib/Battery  Vnom=4.2 V  prm_dir=simscape.enum.battery.prm_dir.disabled  R1_dis=2 Ohm  R1_ch=2 Ohm  R1=0.0065 Ohm  prm_AH=simscape.enum.battery.prm_AH.finite  AH=0.0026 A*hr  V1=3.7 V  AH1=0.00143 A*hr  prm_R2=simscape.enum.battery.prm_R2.disabled  R2=2000 Ohm  Tmeas=298.15 K  charge_measurement_port=simscape.enum.battery.enable.no  prm_dyn=simscape.enum.battery.prm_dyn.off  Rp1=0.005 Ohm  tau1=30 s  Rp2=0.005 Ohm  tau2=30 s  Rp3=0.005 Ohm  tau3=30 s  Rp4=0.005 Ohm  tau4=30 s  Rp5=0.005 Ohm  tau5=30 s  prm_fade=simscape.enum.battery.prm_fade.disabled  N_fade=100  AH_fade=45 A*hr  R1_fade=2.02 Ohm  R1_ch_fade=2.02 Ohm  V1_fade=10.35 V  prm_age=simscape.enum.battery.prm_age.disabled  prm_age_OCV=simscape.enum.battery.prm_age_OCV.OCV  OCV_age=0.9  SOC_age=60  Tmeas_age=298.15 K  delta_time_age_vec=[0] d  temperature_age_vec=[273] K  OCV_scaling_age=2.2134e6  OCV_offset_age=1.632e6  temp_exp_age=0.515833569 V  t_exp_age=0.75  Vnom_T2=12 V  R1_T2=2.2 Ohm  R1_T2_dis=2.2 Ohm  R1_T2_ch=2.2 Ohm  V1_T2=11.4 V  R2_T2=2200 Ohm  Rp1_T2=0.005 Ohm  tau1_T2=30 s  Rp2_T2=0.005 Ohm  tau2_T2=30 s  Rp3_T2=0.005 Ohm  tau3_T2=30 s  Rp4_T2=0.005 Ohm  tau4_T2=30 s  Rp5_T2=0.005 Ohm  tau5_T2=30 s  Tmeas2=273.15 K  thermal_port=simscape.enum.thermaleffects.omit  thermal_mass=30000 J/K  i_specify=off  i_priority=None  i=0 A  i_nominal_specify=off  i_nominal_value=1  i_nominal_unit=A  v_specify=on  v_priority=High  v=3.8 V  v_nominal_specify=off  v_nominal_value=1  v_nominal_unit=V  charge_specify=on  charge_priority=None  charge=0.0026 A*hr  charge_nominal_specify=off  charge_nominal_value=1  charge_nominal_unit=A*hr  num_cycles_specify=off  num_cycles_priority=High  num_cycles=0  num_cycles_nominal_specify=off  num_cycles_nominal_value=1  num_cycles_nominal_unit=1  temperature_specify=off  temperature_priority=High  temperature=298.15 K  temperature_nominal_specify=off  temperature_nominal_value=1  temperature_nominal_unit=K
      settings: LibrarySourceBlock=batt_lib/Cells/Battery
  Battery_Voltage{,1,3..4} (4 alike) : Scope  Commented=on  NumInputPorts=3
      Battery_Voltage settings: ActiveDisplayYMinimum=3.6374983088502764  ActiveDisplayYMaximum=4.2625001879055251  DataLoggingVariableName=ScopeData7
      Battery_Voltage1 settings: ActiveDisplayYMinimum=4.1835535757040772  ActiveDisplayYMaximum=4.1978213168935037  DataLoggingVariableName=ScopeData2
      Battery_Voltage3 settings: ActiveDisplayYMinimum=4.1835535757040772  ActiveDisplayYMaximum=4.1978213168935037  DataLoggingVariableName=ScopeData15
      Battery_Voltage4 settings: ActiveDisplayYMinimum=3.6374983088502764  ActiveDisplayYMaximum=4.2625001879055251  DataLoggingVariableName=ScopeData18
  Battery_Voltage2 : Scope  Commented=on  NumInputPorts=2
      settings: ActiveDisplayYMinimum=3.6374983088502764  ActiveDisplayYMaximum=4.2625001879055251  DataLoggingVariableName=ScopeData11
  Battery_current : Scope  Commented=on  NumInputPorts=5
      settings: ActiveDisplayYMinimum=-0.81813347891934785  ActiveDisplayYMaximum=0.52903090237117911  DataLoggingVariableName=ScopeData8
  Battery_current1 : Scope  Commented=on  NumInputPorts=4
      settings: ActiveDisplayYMinimum=0.71853737193539047  ActiveDisplayYMaximum=1.1980726267735164  DataLoggingVariableName=ScopeData5
  Battery_current2 : Scope  Commented=on  NumInputPorts=5
      settings: ActiveDisplayYMinimum=-0.56854899965387873  ActiveDisplayYMaximum=1.1742832221837642  DataLoggingVariableName=ScopeData12
  Battery_current3 : Scope  Commented=on  NumInputPorts=4
      settings: ActiveDisplayYMinimum=0.71853737193539047  ActiveDisplayYMaximum=1.1980726267735164  DataLoggingVariableName=ScopeData16
  Battery_current4 : Scope  Commented=on  NumInputPorts=5
      settings: ActiveDisplayYMinimum=-0.81813347891934785  ActiveDisplayYMaximum=0.52903090237117911  DataLoggingVariableName=ScopeData19
  Constant : Constant  Commented=on  Value=0.5
  Constant{1,5,7,9} (4 alike) : Constant  Commented=on  Value=0.3
  Constant10 : Constant  Commented=on  Value=0
  Constant11 : Constant  Value=0
  Constant12 : Constant  Value=0.5
  Constant13 : Constant  Value=0.5
  Constant2 : Constant  Commented=on
  Constant3 : Constant  Commented=on  Value=0
  Constant4 : Constant  Commented=on  Value=0
  Constant6 : Constant  Commented=on  Value=0.5
  Constant8 : Constant  Commented=on
  Controlled Current Source{1..5} (5 alike) : fl_lib/Electrical/Electrical Sources/Controlled Current Source  Commented=on
  Controlled Current Source6 : fl_lib/Electrical/Electrical Sources/Controlled Current Source
  Current Sensor{,1..16} (17 alike) : fl_lib/Electrical/Electrical Sensors/Current Sensor  Commented=on
  Current Sensor17 : fl_lib/Electrical/Electrical Sensors/Current Sensor
  Current Sensor18 : fl_lib/Electrical/Electrical Sensors/Current Sensor
  Current Sensor19 : fl_lib/Electrical/Electrical Sensors/Current Sensor
  Data Type Conversion : DataTypeConversion  SaturateOnIntegerOverflow=off  RndMeth=Floor
  Data Type Conversion{1..9} (9 alike) : DataTypeConversion  Commented=on  SaturateOnIntegerOverflow=off  RndMeth=Floor
  Data Type Conversion10 : DataTypeConversion  SaturateOnIntegerOverflow=off  RndMeth=Floor
  Electrical Reference{1..5} (5 alike) : fl_lib/Electrical/Electrical Elements/Electrical Reference  Commented=on
  Electrical Reference6 : fl_lib/Electrical/Electrical Elements/Electrical Reference
  Feedback_BC1 : Subsystem  Commented=on
  Feedback_BC2 : Subsystem  Commented=on
  Feedback_BC3 : Subsystem  Commented=on
  Feedback_BC4 : Subsystem  Commented=on
  Feedback_BC5 : Subsystem  Commented=on
  Feedback_BC6 : Subsystem  Commented=on
  Feedback_BC7 : Subsystem  Commented=on
  Feedback_BC_1 : Subsystem  Commented=on
  Feedback_BC_2 : Subsystem  Commented=on
  From{,1,15..16,32..33,38,41,61..62} (10 alike) : From  Commented=on  GotoTag=V_1  TagVisibility=global
  From{10..11,18..19,34..35,43..44,60,63..64} (11 alike) : From  Commented=on  GotoTag=BC1_IL  TagVisibility=global
  From{12..13,20..21,47..48,65..66} (8 alike) : From  Commented=on  GotoTag=BC2_IL  TagVisibility=global
  From{14,22,49,67} (4 alike) : From  Commented=on  GotoTag=PWM_BC2  TagVisibility=global
  From{17,23,39,50,68} (5 alike) : From  Commented=on  GotoTag=PWM_BC1  TagVisibility=global
  From{2..4,24..26,40,42,51..53,69..71} (14 alike) : From  Commented=on  GotoTag=V_2  TagVisibility=global
  From{5..6,27..28,54..55,72..73} (8 alike) : From  Commented=on  GotoTag=V_3  TagVisibility=global
  From{7,29,45,56,74} (5 alike) : From  Commented=on  GotoTag=I_1  TagVisibility=global
  From{8,30,46,57,75} (5 alike) : From  Commented=on  GotoTag=I_2  TagVisibility=global
  From{9,31,58,76} (4 alike) : From  Commented=on  GotoTag=I_3  TagVisibility=global
  From36 : From  Commented=on  GotoTag=I_bus  TagVisibility=global
  From37 : From  Commented=on  GotoTag=I_bus  TagVisibility=global
  From59 : From  Commented=on  GotoTag=I_bus  TagVisibility=global
  Gain : Gain  Commented=on  Gain=0.1
  Gain1 : Gain  Commented=on  Gain=0.1
  Goto{,10,20,27,39} (5 alike) : Goto  Commented=on  GotoTag=V_1  TagVisibility=global
  Goto{1,11,21,28,40} (5 alike) : Goto  Commented=on  GotoTag=V_2  TagVisibility=global
  Goto{2,12,30,41} (4 alike) : Goto  Commented=on  GotoTag=V_3  TagVisibility=global
  Goto{3,13,23,31,42} (5 alike) : Goto  Commented=on  GotoTag=I_1  TagVisibility=global
  Goto{4,14,24,32,43} (5 alike) : Goto  Commented=on  GotoTag=I_2  TagVisibility=global
  Goto{5,15,33,44} (4 alike) : Goto  Commented=on  GotoTag=I_3  TagVisibility=global
  Goto{6,16,26,34,45} (5 alike) : Goto  Commented=on  GotoTag=BC1_IL  TagVisibility=global
  Goto{7,17,35,46} (4 alike) : Goto  Commented=on  GotoTag=BC2_IL  TagVisibility=global
  Goto{8,18,36,47} (4 alike) : Goto  Commented=on  GotoTag=PWM_BC2  TagVisibility=global
  Goto{9,19,29,37,48} (5 alike) : Goto  Commented=on  GotoTag=PWM_BC1  TagVisibility=global
  Goto22 : Goto  Commented=on  GotoTag=I_bus  TagVisibility=global
  Goto25 : Goto  Commented=on  GotoTag=I_bus  TagVisibility=global
  Goto38 : Goto  Commented=on  GotoTag=I_bus  TagVisibility=global
  Goto49 : Goto  Commented=on  GotoTag=BC1_IL_mea  TagVisibility=global
  I{1..12} (12 alike) : nesl_utility/PS-Simulink Converter  Commented=on  PhysicalDomain=network_engine_domain  SubClassName=ps_output  LeftPortType=input  RightPortType=output  PseudoPeriodic=off  Frequencies=[]  VectorFormat=inherit  Unit=inherit  AffineConversion=off
  I13 : nesl_utility/PS-Simulink Converter  PhysicalDomain=network_engine_domain  SubClassName=ps_output  LeftPortType=input  RightPortType=output  PseudoPeriodic=off  Frequencies=[]  VectorFormat=inherit  Unit=inherit  AffineConversion=off
  I14 : nesl_utility/PS-Simulink Converter  PhysicalDomain=network_engine_domain  SubClassName=ps_output  LeftPortType=input  RightPortType=output  PseudoPeriodic=off  Frequencies=[]  VectorFormat=inherit  Unit=inherit  AffineConversion=off
  I15 : nesl_utility/PS-Simulink Converter  PhysicalDomain=network_engine_domain  SubClassName=ps_output  LeftPortType=input  RightPortType=output  PseudoPeriodic=off  Frequencies=[]  VectorFormat=inherit  Unit=inherit  AffineConversion=off
  I_1 : nesl_utility/PS-Simulink Converter  Commented=on  PhysicalDomain=network_engine_domain  SubClassName=ps_output  LeftPortType=input  RightPortType=output  PseudoPeriodic=off  Frequencies=[]  VectorFormat=inherit  Unit=inherit  AffineConversion=off
  I_2 : nesl_utility/PS-Simulink Converter  Commented=on  PhysicalDomain=network_engine_domain  SubClassName=ps_output  LeftPortType=input  RightPortType=output  PseudoPeriodic=off  Frequencies=[]  VectorFormat=inherit  Unit=inherit  AffineConversion=off
  I_BUS : nesl_utility/PS-Simulink Converter  Commented=on  PhysicalDomain=network_engine_domain  SubClassName=ps_output  LeftPortType=input  RightPortType=output  PseudoPeriodic=off  Frequencies=[]  VectorFormat=inherit  Unit=inherit  AffineConversion=off
  I_BUS1 : nesl_utility/PS-Simulink Converter  Commented=on  PhysicalDomain=network_engine_domain  SubClassName=ps_output  LeftPortType=input  RightPortType=output  PseudoPeriodic=off  Frequencies=[]  VectorFormat=inherit  Unit=inherit  AffineConversion=off
  I_balance : Constant  Commented=on  Value=0.3
  I_balance1 : Constant  Commented=on  Value=0.3
  I_balance2 : Constant  Commented=on  Value=0.3
  I_battery2 : Display
  I_battery3 : Display
  I_bus : nesl_utility/PS-Simulink Converter  Commented=on  PhysicalDomain=network_engine_domain  SubClassName=ps_output  LeftPortType=input  RightPortType=output  PseudoPeriodic=off  Frequencies=[]  VectorFormat=inherit  Unit=inherit  AffineConversion=off
  Lambda_BC1 : Subsystem  Commented=on
  Lambda_BC2 : Subsystem  Commented=on
  Lambda_BC3 : Subsystem  Commented=on
  Lambda_BC4 : Subsystem  Commented=on
  Lambda_BC5 : Subsystem  Commented=on
  Lambda_BC6 : Subsystem  Commented=on
  Lambda_BC7 : Subsystem  Commented=on
  Lambda_BC8 : Subsystem  Commented=on
  Lambda_BC9 : Subsystem  Commented=on
  Moving Average{,1..25} (26 alike) : eeGeneralControl/Moving Average  Commented=on  VariantControl=Variant1  LabelModeActiveChoice=Discrete  f=1e5  x0=0  BufferSize=8192  Ts=1e-7
      settings: LibrarySourceBlock=ee_sl_lib/General Control/Moving Average
  NOT{,1..8} (9 alike) : Logic  Commented=on  Operator=NOT  IconShape=distinctive  AllPortsSameDT=off  OutDataTypeStr=boolean
  NOT10 : Logic  Operator=NOT  IconShape=distinctive  AllPortsSameDT=off  OutDataTypeStr=boolean
  NOT9 : Logic  Operator=NOT  IconShape=distinctive  AllPortsSameDT=off  OutDataTypeStr=boolean
  PWM : simulink/Discontinuities/PWM  DisableCoverage=on  Period=1e-6  InitialDelay=0  DisallowZeroDutyCycle=off  RunAtFixedTimeIntervals=off  SampleTime=0.1
  PWM Generator : eePwmGenerator/PWM Generator  Commented=on  CarrCount=Up  Tper=4  Tdelay=0  Ts=0.1
  PWM Generator1 : eePwmGenerator/PWM Generator  Commented=on  CarrCount=Up  Tper=4  Tdelay=0  Ts=0.1
  PWM1 : simulink/Discontinuities/PWM  DisableCoverage=on  Period=1e-6  InitialDelay=0  DisallowZeroDutyCycle=off  RunAtFixedTimeIntervals=off  SampleTime=0.1
  Product{,1..8} (9 alike) : Product  Commented=on  Inputs=3
  Scope : Scope  NumInputPorts=5
      settings: ActiveDisplayYMinimum=-4.421959989881322E-5  ActiveDisplayYMaximum=7.3540474441577663E-5  DataLoggingVariableName=ScopeData20
  Simulink-PS Converter{1,5,11,14,19} (5 alike) : nesl_utility/Simulink-PS Converter  Commented=on  PhysicalDomain=network_engine_domain  SubClassName=ps_input  LeftPortType=input  RightPortType=output  PseudoPeriodic=off  Frequencies=[]  NoiseDistribution=none  NoiseParameters=[]  Unit=1  AffineConversion=off  FilteringAndDerivatives=provide  SimscapeFilterOrder=1  InputFilterTimeConstant=0.001  UdotUserProvided=0
  Simulink-PS Converter{2..4,6..10,12..13,15..18,20..23} (18 alike) : nesl_utility/Simulink-PS Converter  Commented=on  PhysicalDomain=network_engine_domain  SubClassName=ps_input  LeftPortType=input  RightPortType=output  PseudoPeriodic=off  Frequencies=[]  NoiseDistribution=none  NoiseParameters=[]  Unit=1  AffineConversion=off  FilteringAndDerivatives=zero  SimscapeFilterOrder=1  InputFilterTimeConstant=0.001  UdotUserProvided=0
  Simulink-PS Converter24 : nesl_utility/Simulink-PS Converter  PhysicalDomain=network_engine_domain  SubClassName=ps_input  LeftPortType=input  RightPortType=output  PseudoPeriodic=off  Frequencies=[]  NoiseDistribution=none  NoiseParameters=[]  Unit=1  AffineConversion=off  FilteringAndDerivatives=provide  SimscapeFilterOrder=1  InputFilterTimeConstant=0.001  UdotUserProvided=0
  Simulink-PS Converter{25..28} (4 alike) : nesl_utility/Simulink-PS Converter  PhysicalDomain=network_engine_domain  SubClassName=ps_input  LeftPortType=input  RightPortType=output  PseudoPeriodic=off  Frequencies=[]  NoiseDistribution=none  NoiseParameters=[]  Unit=1  AffineConversion=off  FilteringAndDerivatives=zero  SimscapeFilterOrder=1  InputFilterTimeConstant=0.001  UdotUserProvided=0
  Solver Configuration{1..5} (5 alike) : nesl_utility/Solver Configuration  Commented=on  PhysicalDomain=network_engine_domain  SubClassName=solver  LeftPortType=input  RightPortType=generic  Tones=[]  Harmonics=[]  SimulateNoise=off  Profile=off  UseLocalSampling=off  EnableSwitchedLinearOptims=on  FrequencyDomain=off  UseCCode=off  RelTol=0.001  AbsTol=0.001  MinStep=1e-09  ToWorkspace=off  RevertToSquareIcSolve=off  NumHomotopyIterations=100  PhasorMode=off  PhasorModeNumHarmonics=1  ConsistencySolver=NEWTON_XTOL_AFTER_FTOL  IndexReductionMethod=DerivativeReplacement  DoDC=off  ResidualTolerance=1e-09  ConsistencyTolSource=GLOBAL  ConsistencyAbsTol=0.001  ConsistencyRelTol=0.001  ConsistencyTolFactor=0.001  UseLocalSolver=on  LocalSolverChoice=NE_BACKWARD_EULER_ADVANCER  ResolveIndetEquations=on  FunctionEvalNumThread=1  LocalSolverSampleTime=1e-6  DoFixedCost=off  MaxNonlinIter=3  MaxModeIter=2  ComputeImpulses=off  ImpulseIterations=2  LinearAlgebra=auto  LinearAlgebraNumThread=0  EquationFormulation=NE_TIME_EF  DelaysMemoryBudget=1024  AutomaticFiltering=on  FilteringTimeConstant=0.001  PartitionStorageMethod=AS_NEEDED  PartitionMemoryBudget=1024  PartitionMethod=ROBUST  MultibodyUseLocalSolver=off  MultibodyLocalSolverChoice=ODE1  MultibodyLocalSolverSampleTime=0.001
  Solver Configuration6 : nesl_utility/Solver Configuration  PhysicalDomain=network_engine_domain  SubClassName=solver  LeftPortType=input  RightPortType=generic  Tones=[]  Harmonics=[]  SimulateNoise=off  Profile=off  UseLocalSampling=off  EnableSwitchedLinearOptims=on  FrequencyDomain=off  UseCCode=off  RelTol=0.001  AbsTol=0.001  MinStep=1e-09  ToWorkspace=off  RevertToSquareIcSolve=off  NumHomotopyIterations=100  PhasorMode=off  PhasorModeNumHarmonics=1  ConsistencySolver=NEWTON_XTOL_AFTER_FTOL  IndexReductionMethod=DerivativeReplacement  DoDC=off  ResidualTolerance=1e-09  ConsistencyTolSource=GLOBAL  ConsistencyAbsTol=0.001  ConsistencyRelTol=0.001  ConsistencyTolFactor=0.001  UseLocalSolver=on  LocalSolverChoice=NE_BACKWARD_EULER_ADVANCER  ResolveIndetEquations=on  FunctionEvalNumThread=1  LocalSolverSampleTime=2e-8  DoFixedCost=off  MaxNonlinIter=3  MaxModeIter=2  ComputeImpulses=off  ImpulseIterations=2  LinearAlgebra=auto  LinearAlgebraNumThread=0  EquationFormulation=NE_TIME_EF  DelaysMemoryBudget=1024  AutomaticFiltering=on  FilteringTimeConstant=0.001  PartitionStorageMethod=AS_NEEDED  PartitionMemoryBudget=1024  PartitionMethod=ROBUST  MultibodyUseLocalSolver=off  MultibodyLocalSolverChoice=ODE1  MultibodyLocalSolverSampleTime=0.001
  Sum : Sum  Commented=on  Inputs=|++
  Sum{1..9,11..19} (18 alike) : Sum  Commented=on  Inputs=|+-
  Sum10 : Sum  Commented=on  Inputs=|++
  V1 : nesl_utility/PS-Simulink Converter  Commented=on  PhysicalDomain=network_engine_domain  SubClassName=ps_output  LeftPortType=input  RightPortType=output  PseudoPeriodic=off  Frequencies=[]  VectorFormat=inherit  Unit=inherit  AffineConversion=off
  V2 : nesl_utility/PS-Simulink Converter  Commented=on  PhysicalDomain=network_engine_domain  SubClassName=ps_output  LeftPortType=input  RightPortType=output  PseudoPeriodic=off  Frequencies=[]  VectorFormat=inherit  Unit=inherit  AffineConversion=off
  V_{1..12} (12 alike) : nesl_utility/PS-Simulink Converter  Commented=on  PhysicalDomain=network_engine_domain  SubClassName=ps_output  LeftPortType=input  RightPortType=output  PseudoPeriodic=off  Frequencies=[]  VectorFormat=inherit  Unit=inherit  AffineConversion=off
  V_13 : nesl_utility/PS-Simulink Converter  PhysicalDomain=network_engine_domain  SubClassName=ps_output  LeftPortType=input  RightPortType=output  PseudoPeriodic=off  Frequencies=[]  VectorFormat=inherit  Unit=inherit  AffineConversion=off
  V_14 : nesl_utility/PS-Simulink Converter  PhysicalDomain=network_engine_domain  SubClassName=ps_output  LeftPortType=input  RightPortType=output  PseudoPeriodic=off  Frequencies=[]  VectorFormat=inherit  Unit=inherit  AffineConversion=off
  V_15 : nesl_utility/PS-Simulink Converter  PhysicalDomain=network_engine_domain  SubClassName=ps_output  LeftPortType=input  RightPortType=output  PseudoPeriodic=off  Frequencies=[]  VectorFormat=inherit  Unit=inherit  AffineConversion=off
  Voltage Sensor{1..14} (14 alike) : fl_lib/Electrical/Electrical Sensors/Voltage Sensor  Commented=on
  Voltage Sensor15 : fl_lib/Electrical/Electrical Sensors/Voltage Sensor
  Voltage Sensor16 : fl_lib/Electrical/Electrical Sensors/Voltage Sensor
  Voltage Sensor17 : fl_lib/Electrical/Electrical Sensors/Voltage Sensor
  iL_1 : Display
  iL_2 : Display
  tag scope: BC1_IL=global, BC2_IL=global, I_1=global, I_2=global, I_3=global, V_1=global, V_2=global, V_3=global
  wires:
  Constant3/1 -> Simulink-PS Converter5/1
  Alpha1/1(alpha1) -> Product/3
  I_balance/1 -> Product/1, Product1/3
  Product/1 -> Sum6/1  "I_ref1"
  Alpha2/1(alpha2) -> Product1/2
  Product1/1 -> Sum5/1  "I_ref2"
  NOT1/1 -> Data Type Conversion1/1
  NOT/1 -> Data Type Conversion2/1
  Moving Average1/1 -> Sum6/2  "BC1_IL_mea"
  Moving Average/1 -> Sum5/2  "BC2_IL_mea"
  Moving Average2/1 -> Alpha2/1(V32), Lambda_BC2/1(In1)
  Moving Average3/1 -> Alpha1/1(V21), Lambda_BC1/1(In1)
  Sum2/1 -> Moving Average3/1  "V21"
  Sum3/1 -> Moving Average2/1  "V32"
  Sum6/1 -> Feedback_BC1/1(u)
  Sum5/1 -> Feedback_BC2/1(u)
  Lambda_BC2/1(Lambda_BC2) -> Product1/1
  From/1 -> Battery_Voltage/3
  From1/1 -> Sum2/2
  V_1/1 -> Goto/1
  From2/1 -> Battery_Voltage/2
  From4/1 -> Sum2/1
  From3/1 -> Sum3/2
  V_2/1 -> Goto1/1
  From5/1 -> Sum3/1
  From6/1 -> Battery_Voltage/1
  V_3/1 -> Goto2/1
  I3/1 -> Goto3/1
  From7/1 -> Battery_current/3
  I2/1 -> Goto4/1
  From8/1 -> Battery_current/2
  I1/1 -> Goto5/1
  From9/1 -> Battery_current/1
  From10/1 -> Moving Average1/1
  From11/1 -> BC_IL/2
  BC1_IL/1 -> Goto6/1
  From12/1 -> BC_IL/1
  From13/1 -> Moving Average/1
  BC2_IL/1 -> Goto7/1
  Lambda_BC1/1(Lambda_BC1) -> Product/2
  Data Type Conversion2/1 -> Simulink-PS Converter7/1
  From17/1 -> Simulink-PS Converter6/1, NOT/1
  Data Type Conversion1/1 -> Simulink-PS Converter9/1
  From14/1 -> Simulink-PS Converter8/1, NOT1/1
  Constant/1 -> PWM Generator/1
  PWM Generator/1 -> Gain/1
  Gain/1 -> Sum/1
  Constant1/1 -> Sum/2
  From24/1 -> Battery_Voltage1/2
  Product2/1 -> Sum8/1  "I_ref1"
  From19/1 -> BC_IL1/2
  Lambda_BC3/1(Lambda_BC1) -> Product2/2
  Moving Average4/1 -> Sum7/2  "BC2_IL_mea"
  Sum1/1 -> Moving Average7/1  "V21"
  Data Type Conversion4/1 -> Simulink-PS Converter3/1
  From27/1 -> Sum4/1
  Feedback_BC3/1(PWM) -> Goto19/1
  From28/1 -> Battery_Voltage1/1
  From25/1 -> Sum4/2
  NOT2/1 -> Data Type Conversion4/1
  Constant2/1 -> Simulink-PS Converter1/1
  From16/1 -> Sum1/2
  From22/1 -> Simulink-PS Converter4/1, NOT3/1
  Moving Average5/1 -> Sum8/2  "BC1_IL_mea"
  NOT3/1 -> Data Type Conversion3/1
  I4/1 -> Goto15/1
  Product3/1 -> Sum7/1  "I_ref2"
  From29/1 -> Moving Average12/1
  From26/1 -> Sum1/1
  From18/1 -> Moving Average5/1
  Moving Average6/1 -> Alpha4/1(V32), Lambda_BC4/1(In1)
  I5/1 -> Goto14/1
  From30/1 -> Moving Average10/1
  Sum7/1 -> Feedback_BC_2/1(u)
  Sum4/1 -> Moving Average6/1  "V32"
  Moving Average7/1 -> Alpha3/1(V21), Lambda_BC3/1(In1)
  From31/1 -> Moving Average8/1
  Sum8/1 -> Feedback_BC3/1(u)
  Alpha4/1(alpha2) -> Product3/2
  From21/1 -> Moving Average4/1
  Lambda_BC4/1(Lambda_BC2) -> Product3/1
  Feedback_BC_2/1(PWM) -> Goto18/1
  From15/1 -> Battery_Voltage1/3
  Alpha3/1(alpha1) -> Product2/3
  From23/1 -> Simulink-PS Converter2/1, NOT2/1
  BC2_IL1/1 -> Goto17/1
  From20/1 -> BC_IL1/1
  Data Type Conversion3/1 -> Simulink-PS Converter10/1
  V_5/1 -> Goto11/1
  BC1_IL1/1 -> Goto16/1
  V_6/1 -> Goto12/1
  I6/1 -> Goto13/1
  V_4/1 -> Goto10/1
  From40/1 -> Battery_Voltage2/1
  Product4/1 -> Sum12/1  "I_ref1"
  From35/1 -> BC_IL2/1
  Lambda_BC5/1(Lambda_BC1) -> Product4/2
  Sum9/1 -> Moving Average11/1  "V21"
  Data Type Conversion6/1 -> Simulink-PS Converter13/1
  Feedback_BC5/1(PWM) -> Battery_current2/5, Goto29/1
  NOT4/1 -> Data Type Conversion6/1
  Constant4/1 -> Simulink-PS Converter11/1
  From33/1 -> Sum9/2
  Moving Average9/1 -> Sum12/2  "BC1_IL_mea"
  From45/1 -> Battery_current2/3
  From42/1 -> Sum9/1
  From34/1 -> Moving Average9/1
  I_2/1 -> Goto24/1
  From46/1 -> Battery_current2/2
  Moving Average11/1 -> Alpha5/1(V21), Lambda_BC5/1(In1)
  From36/1 -> Battery_current2/1
  Sum12/1 -> Feedback_BC5/1(u)
  From32/1 -> Battery_Voltage2/2
  Alpha5/1(alpha1) -> Product4/3
  From39/1 -> Simulink-PS Converter12/1, NOT4/1
  V2/1 -> Goto21/1
  BC1_IL2/1 -> Goto26/1
  I_balance1/1 -> Product4/1
  I_1/1 -> Goto23/1
  V1/1 -> Goto20/1
  I_bus/1 -> Goto22/1
  I_BUS/1 -> Goto25/1
  From37/1 -> Moving Average13/1
  Constant5/1 -> Product2/1, Product3/3
  Moving Average8/1 -> Battery_current1/1  "I3_mean"
  Moving Average10/1 -> Battery_current1/2  "I2_mean"
  Moving Average12/1 -> Battery_current1/3  "I1_mean"
  Moving Average13/1 -> Battery_current1/4  "I_bus_mean"
  Feedback_BC_1/1(PWM) -> Goto36/1
  BC2_IL2/1 -> Goto35/1
  From51/1 -> Battery_Voltage3/2
  From43/1 -> Moving Average18/1
  From58/1 -> Moving Average21/1
  Constant9/1 -> Product5/1, Product6/3
  PWM Generator1/1 -> Gain1/1
  V_7/1 -> Goto27/1
  Feedback_BC4/1(PWM) -> Goto37/1
  Sum13/1 -> Moving Average19/1  "V32"
  V_9/1 -> Goto30/1
  Data Type Conversion7/1 -> Simulink-PS Converter17/1
  Moving Average19/1 -> Alpha7/1(V32), Lambda_BC7/1(In1)
  From47/1 -> BC_IL3/1
  Moving Average18/1 -> Sum15/2  "BC1_IL_mea"
  Moving Average21/1 -> Battery_current3/1  "I3_mean"
  Moving Average20/1 -> Alpha6/1(V21), Lambda_BC6/1(In1)
  V_8/1 -> Goto28/1
  I8/1 -> Goto32/1
  NOT6/1 -> Data Type Conversion5/1
  Moving Average15/1 -> Battery_current3/3  "I1_mean"
  Sum11/1 -> Moving Average20/1  "V21"
  Lambda_BC7/1(Lambda_BC2) -> Product6/1
  From56/1 -> Moving Average15/1
  Sum15/1 -> Feedback_BC4/1(u)
  Sum14/1 -> Feedback_BC_1/1(u)
  Product5/1 -> Sum15/1  "I_ref1"
  From57/1 -> Moving Average14/1
  From53/1 -> Sum11/1
  From41/1 -> Sum11/2
  From44/1 -> BC_IL3/2
  From38/1 -> Battery_Voltage3/3
  Lambda_BC6/1(Lambda_BC1) -> Product5/2
  From59/1 -> Moving Average16/1
  NOT5/1 -> Data Type Conversion7/1
  Gain1/1 -> Sum10/1
  From55/1 -> Battery_Voltage3/1
  From50/1 -> Simulink-PS Converter16/1, NOT5/1
  From49/1 -> Simulink-PS Converter18/1, NOT6/1
  Alpha6/1(alpha1) -> Product5/3
  Moving Average16/1 -> Battery_current3/4  "I_bus_mean"
  Product6/1 -> Sum14/1  "I_ref2"
  From52/1 -> Sum13/2
  Constant7/1 -> Sum10/2
  Alpha7/1(alpha2) -> Product6/2
  Moving Average14/1 -> Battery_current3/2  "I2_mean"
  Constant8/1 -> Simulink-PS Converter14/1
  I_BUS1/1 -> Goto38/1
  I9/1 -> Goto31/1
  Constant6/1 -> PWM Generator1/1
  BC1_IL3/1 -> Goto34/1
  From54/1 -> Sum13/1
  Moving Average17/1 -> Sum14/2  "BC2_IL_mea"
  I7/1 -> Goto33/1
  Data Type Conversion5/1 -> Simulink-PS Converter15/1
  From48/1 -> Moving Average17/1
  From60/1 -> Battery_current2/4
  Feedback_BC1/1(PWM) -> Goto9/1, Battery_current/4
  Feedback_BC2/1(PWM) -> Goto8/1, Battery_current/5
  From69/1 -> Battery_Voltage4/2
  From67/1 -> Simulink-PS Converter22/1, NOT8/1
  I_balance2/1 -> Product7/1, Product8/3
  Sum18/1 -> Feedback_BC7/1(u)
  Lambda_BC8/1(Lambda_BC1) -> Product7/2
  BC1_IL4/1 -> Goto45/1
  Moving Average23/1 -> Goto49/1, Sum19/2  "BC1_IL_mea"
  Sum19/1 -> Feedback_BC6/1(u)
  From65/1 -> BC_IL4/1
  From61/1 -> Battery_Voltage4/3
  From66/1 -> Moving Average22/1
  Data Type Conversion9/1 -> Simulink-PS Converter21/1
  From73/1 -> Battery_Voltage4/1
  From72/1 -> Sum17/1
  V_10/1 -> Goto39/1
  Product7/1 -> Sum19/1  "I_ref1"
  Data Type Conversion8/1 -> Simulink-PS Converter23/1
  I12/1 -> Goto42/1
  BC2_IL3/1 -> Goto46/1
  Alpha8/1(alpha1) -> Product7/3
  From71/1 -> Sum16/1
  Sum16/1 -> Moving Average25/1  "V21"
  Constant10/1 -> Simulink-PS Converter19/1
  From64/1 -> BC_IL4/2
  From74/1 -> Battery_current4/3
  Alpha9/1(alpha2) -> Product8/2
  From76/1 -> Battery_current4/1
  NOT8/1 -> Data Type Conversion8/1
  Moving Average22/1 -> Sum18/2  "BC2_IL_mea"
  V_11/1 -> Goto40/1
  V_12/1 -> Goto41/1
  From70/1 -> Sum17/2
  Moving Average25/1 -> Alpha8/1(V21), Lambda_BC8/1(In1)
  I11/1 -> Goto43/1
  From68/1 -> Simulink-PS Converter20/1, NOT7/1
  Moving Average24/1 -> Alpha9/1(V32), Lambda_BC9/1(In1)
  Feedback_BC6/1(PWM) -> Goto48/1, Battery_current4/4
  Lambda_BC9/1(Lambda_BC2) -> Product8/1
  NOT7/1 -> Data Type Conversion9/1
  From75/1 -> Battery_current4/2
  From63/1 -> Moving Average23/1
  Product8/1 -> Sum18/1  "I_ref2"
  Sum17/1 -> Moving Average24/1  "V32"
  I10/1 -> Goto44/1
  From62/1 -> Sum16/2
  Feedback_BC7/1(PWM) -> Goto47/1, Battery_current4/5
  I14/1 -> [I_2]
  BC2_IL4/1 -> [BC2_IL]
  Constant12/1 -> PWM/1
  I13/1 -> [I_3]
  BC1_IL5/1 -> [BC1_IL]
  V_14/1 -> [V_2]
  I15/1 -> [I_1]
  Constant11/1 -> Simulink-PS Converter24/1
  V_13/1 -> [V_1]
  Constant13/1 -> PWM1/1
  V_15/1 -> [V_3]
  [I_1] -> Scope/3
  [BC1_IL] -> iL_1/1, Scope/1
  [BC2_IL] -> iL_2/1, Scope/2
  [I_2] -> I_battery2/1, Scope/4
  [I_3] -> I_battery3/1, Scope/5
  PWM/1 -> Simulink-PS Converter27/1, NOT9/1
  NOT9/1 -> Data Type Conversion/1
  Data Type Conversion/1 -> Simulink-PS Converter28/1
  PWM1/1 -> Simulink-PS Converter25/1, NOT10/1
  NOT10/1 -> Data Type Conversion10/1
  Data Type Conversion10/1 -> Simulink-PS Converter26/1
  connections:
  Voltage Sensor3/RConn2 -- Battery _1/RConn1 -- Electrical Reference1/LConn1 -- Solver Configuration1/RConn1 -- Controlled Current Source1/LConn1 -- BC1/LConn3
  BC1/LConn1 -- Battery _3/RConn1 -- Voltage Sensor5/RConn2 -- BC2/LConn2 -- Current Sensor4/RConn2
  Voltage Sensor4/RConn2 -- BC2/LConn3 -- Current Sensor5/RConn2 -- Battery _2/RConn1 -- BC1/LConn2
  Current Sensor4/LConn1 -- Battery _2/LConn1 -- Voltage Sensor4/LConn1
  Current Sensor3/LConn1 -- Battery _3/LConn1 -- Voltage Sensor5/LConn1
  Current Sensor3/RConn2 -- BC2/LConn1 -- Controlled Current Source1/RConn2
  Current Sensor5/LConn1 -- Battery _1/LConn1 -- Voltage Sensor3/LConn1
  Current Sensor3/RConn1 -- I1/LConn1
  Simulink-PS Converter8/RConn1 -- BC2/RConn1
  Simulink-PS Converter9/RConn1 -- BC2/RConn2
  Simulink-PS Converter7/RConn1 -- BC1/RConn2
  Simulink-PS Converter6/RConn1 -- BC1/RConn1
  V_1/LConn1 -- Voltage Sensor3/RConn1
  BC2_IL/LConn1 -- BC2/RConn3
  V_2/LConn1 -- Voltage Sensor4/RConn1
  BC1_IL/LConn1 -- BC1/RConn3
  Simulink-PS Converter5/RConn1 -- Controlled Current Source1/RConn1
  V_3/LConn1 -- Voltage Sensor5/RConn1
  Current Sensor5/RConn1 -- I3/LConn1
  Current Sensor4/RConn1 -- I2/LConn1
  BC_2/LConn2 -- BC_1/LConn1 -- Battery 3/RConn1 -- Current Sensor2/RConn2 -- Voltage Sensor6/RConn2
  BC_2/LConn1 -- Current Sensor7/LConn1 -- Current Sensor1/RConn2
  Voltage Sensor6/LConn1 -- Current Sensor1/LConn1 -- Battery 3/LConn1
  Voltage Sensor2/LConn1 -- Current Sensor2/LConn1 -- Battery 2/LConn1
  BC_1/LConn2 -- Voltage Sensor2/RConn2 -- BC_2/LConn3 -- Current Sensor6/RConn2 -- Battery 2/RConn1
  Voltage Sensor1/LConn1 -- Current Sensor6/LConn1 -- Battery 1/LConn1
  Controlled Current Source2/LConn1 -- Solver Configuration2/RConn1 -- Voltage Sensor1/RConn2 -- BC_1/LConn3 -- Battery 1/RConn1 -- Electrical Reference2/LConn1
  Current Sensor6/RConn1 -- I6/LConn1
  BC1_IL1/LConn1 -- BC_1/RConn3
  V_4/LConn1 -- Voltage Sensor1/RConn1
  Current Sensor2/RConn1 -- I5/LConn1
  BC2_IL1/LConn1 -- BC_2/RConn3
  Simulink-PS Converter4/RConn1 -- BC_2/RConn1
  Simulink-PS Converter1/RConn1 -- Controlled Current Source2/RConn1
  Simulink-PS Converter2/RConn1 -- BC_1/RConn1
  V_6/LConn1 -- Voltage Sensor6/RConn1
  V_5/LConn1 -- Voltage Sensor2/RConn1
  Current Sensor1/RConn1 -- I4/LConn1
  Simulink-PS Converter10/RConn1 -- BC_2/RConn2
  Simulink-PS Converter3/RConn1 -- BC_1/RConn2
  Voltage Sensor8/LConn1 -- Current Sensor8/LConn1 -- Battery 2_/LConn1
  BC5/LConn2 -- Voltage Sensor8/RConn2 -- Current Sensor9/RConn2 -- Battery 2_/RConn1
  Voltage Sensor7/LConn1 -- Current Sensor9/LConn1 -- Battery 1_/LConn1
  Controlled Current Source3/LConn1 -- Solver Configuration3/RConn1 -- Voltage Sensor7/RConn2 -- BC5/LConn3 -- Battery 1_/RConn1 -- Electrical Reference3/LConn1
  Current Sensor9/RConn1 -- I_1/LConn1
  BC1_IL2/LConn1 -- BC5/RConn3
  Simulink-PS Converter13/RConn1 -- BC5/RConn2
  V1/LConn1 -- Voltage Sensor7/RConn1
  Current Sensor8/RConn1 -- I_2/LConn1
  Simulink-PS Converter12/RConn1 -- BC5/RConn1
  V2/LConn1 -- Voltage Sensor8/RConn1
  Simulink-PS Converter11/RConn1 -- Controlled Current Source3/RConn1
  BC5/LConn1 -- Current Sensor/LConn1 -- Current Sensor8/RConn2
  I_bus/LConn1 -- Current Sensor/RConn1
  Current Sensor/RConn2 -- Controlled Current Source3/RConn2
  Current Sensor7/RConn2 -- Controlled Current Source2/RConn2
  I_BUS/LConn1 -- Current Sensor7/RConn1
  Voltage Sensor11/RConn2 -- BC_4/LConn2 -- BC_3/LConn1 -- Battery 6/RConn1 -- Current Sensor11/RConn2
  Battery 4/RConn1 -- Controlled Current Source4/LConn1 -- Solver Configuration4/RConn1 -- Electrical Reference4/LConn1 -- Voltage Sensor9/RConn2 -- BC_3/LConn3
  Current Sensor10/RConn2 -- BC_4/LConn1 -- Current Sensor13/LConn1
  BC_4/LConn3 -- BC_3/LConn2 -- Current Sensor12/RConn2 -- Battery 5/RConn1 -- Voltage Sensor10/RConn2
  Battery 5/LConn1 -- Voltage Sensor10/LConn1 -- Current Sensor11/LConn1
  Battery 4/LConn1 -- Voltage Sensor9/LConn1 -- Current Sensor12/LConn1
  Battery 6/LConn1 -- Voltage Sensor11/LConn1 -- Current Sensor10/LConn1
  V_8/LConn1 -- Voltage Sensor10/RConn1
  Simulink-PS Converter17/RConn1 -- BC_3/RConn2
  Simulink-PS Converter14/RConn1 -- Controlled Current Source4/RConn1
  Simulink-PS Converter16/RConn1 -- BC_3/RConn1
  V_9/LConn1 -- Voltage Sensor11/RConn1
  V_7/LConn1 -- Voltage Sensor9/RConn1
  Current Sensor10/RConn1 -- I7/LConn1
  Current Sensor11/RConn1 -- I8/LConn1
  Current Sensor12/RConn1 -- I9/LConn1
  Current Sensor13/RConn2 -- Controlled Current Source4/RConn2
  BC2_IL2/LConn1 -- BC_4/RConn3
  Simulink-PS Converter18/RConn1 -- BC_4/RConn1
  I_BUS1/LConn1 -- Current Sensor13/RConn1
  BC1_IL3/LConn1 -- BC_3/RConn3
  Simulink-PS Converter15/RConn1 -- BC_4/RConn2
  BC4/LConn2 -- BC3/LConn1 -- Battery _6/RConn1 -- Current Sensor15/RConn2 -- Voltage Sensor14/RConn2
  Controlled Current Source5/LConn1 -- Voltage Sensor12/RConn2 -- BC3/LConn3 -- Battery _4/RConn1 -- Electrical Reference5/LConn1 -- Solver Configuration5/RConn1
  Voltage Sensor12/LConn1 -- Current Sensor16/LConn1 -- Battery _4/LConn1
  Voltage Sensor13/LConn1 -- Current Sensor15/LConn1 -- Battery _5/LConn1
  BC3/LConn2 -- Current Sensor16/RConn2 -- Battery _5/RConn1 -- Voltage Sensor13/RConn2 -- BC4/LConn3
  Voltage Sensor14/LConn1 -- Current Sensor14/LConn1 -- Battery _6/LConn1
  Controlled Current Source5/RConn2 -- Current Sensor14/RConn2 -- BC4/LConn1
  Simulink-PS Converter21/RConn1 -- BC3/RConn2
  Current Sensor15/RConn1 -- I11/LConn1
  BC2_IL3/LConn1 -- BC4/RConn3
  V_11/LConn1 -- Voltage Sensor13/RConn1
  Current Sensor16/RConn1 -- I12/LConn1
  Simulink-PS Converter22/RConn1 -- BC4/RConn1
  V_10/LConn1 -- Voltage Sensor12/RConn1
  Simulink-PS Converter23/RConn1 -- BC4/RConn2
  BC1_IL4/LConn1 -- BC3/RConn3
  Simulink-PS Converter19/RConn1 -- Controlled Current Source5/RConn1
  V_12/LConn1 -- Voltage Sensor14/RConn1
  Simulink-PS Converter20/RConn1 -- BC3/RConn1
  Current Sensor14/RConn1 -- I10/LConn1
  Battery _9/LConn1 -- Voltage Sensor17/LConn1 -- Current Sensor17/LConn1
  Voltage Sensor17/RConn2 -- BC7/LConn2 -- BC6/LConn1 -- Battery _9/RConn1 -- Current Sensor18/RConn2
  Battery _7/LConn1 -- Voltage Sensor15/LConn1 -- Current Sensor19/LConn1
  Battery _7/RConn1 -- Controlled Current Source6/LConn1 -- Solver Configuration6/RConn1 -- Electrical Reference6/LConn1 -- Voltage Sensor15/RConn2 -- BC6/LConn3
  BC7/LConn1 -- Controlled Current Source6/RConn2 -- Current Sensor17/RConn2
  BC7/LConn3 -- Voltage Sensor16/RConn2 -- BC6/LConn2 -- Current Sensor19/RConn2 -- Battery _8/RConn1
  Battery _8/LConn1 -- Voltage Sensor16/LConn1 -- Current Sensor18/LConn1
  BC2_IL4/LConn1 -- BC7/RConn3
  Simulink-PS Converter28/RConn1 -- BC7/RConn2
  V_15/LConn1 -- Voltage Sensor17/RConn1
  Simulink-PS Converter27/RConn1 -- BC7/RConn1
  BC1_IL5/LConn1 -- BC6/RConn3
  Simulink-PS Converter26/RConn1 -- BC6/RConn2
  Current Sensor18/RConn1 -- I14/LConn1
  Current Sensor17/RConn1 -- I13/LConn1
  V_14/LConn1 -- Voltage Sensor16/RConn1
  Simulink-PS Converter25/RConn1 -- BC6/RConn1
  Simulink-PS Converter24/RConn1 -- Controlled Current Source6/RConn1
  V_13/LConn1 -- Voltage Sensor15/RConn1
  Current Sensor19/RConn1 -- I15/LConn1
